simulink model "model"  (R2014a)
(part 2 of 3)

  _CN_244062688_500000_CN_163913701_500000 : powerlib/Elements/Distributed Parameters Line  Phases=3  Frequency=60  Resistance=[0.01273 0.3864]  Inductance="[0.9337e-3  4.1264e-3]"  Capacitance=[12.74e-9 7.751e-9]  Length=114.838  x1=[0 0 0 0; 0.0001244 0 0 0; 0.0002488 0 0 0; 0.0003733 0 0 0; 0.0004977 0 0 0; 0.0006221 0 0 0]  x2=[0 0 0 0; 0.0001244 0 0 0; 0.0002488 0 0 0; 0.0003733 0 0 0; 0.0004977 0 0 0; 0.0006221 0 0 0]  x3=[0 0 0 0; 0.0001244 0 0 0; 0.0002488 0 0 0; 0.0003733 0 0 0; 0.0004977 0 0 0; 0.0006221 0 0 0]  x4=[0 0 0 0; 0.0001244 0 0 0; 0.0002488 0 0 0; 0.0003733 0 0 0; 0.0004977 0 0 0; 0.0006221 0 0 0]  x5=0  V1=ones(3,3)  V2=ones(3,3)  I1=ones(3,3)  I2=ones(3,3)  nHarmo=1  Measurements=None
  _CN_255032299_110000_CN_255032301_110000 : powerlib/Elements/Distributed Parameters Line  Phases=3  Frequency=60  Resistance=[0.01273 0.3864]  Inductance="[0.9337e-3  4.1264e-3]"  Capacitance=[12.74e-9 7.751e-9]  Length=20.7716  x1=[0 0 0 0; 0.0001244 0 0 0; 0.0002488 0 0 0; 0.0003733 0 0 0; 0.0004977 0 0 0; 0.0006221 0 0 0]  x2=[0 0 0 0; 0.0001244 0 0 0; 0.0002488 0 0 0; 0.0003733 0 0 0; 0.0004977 0 0 0; 0.0006221 0 0 0]  x3=[0 0 0 0; 0.0001244 0 0 0; 0.0002488 0 0 0; 0.0003733 0 0 0; 0.0004977 0 0 0; 0.0006221 0 0 0]  x4=[0 0 0 0; 0.0001244 0 0 0; 0.0002488 0 0 0; 0.0003733 0 0 0; 0.0004977 0 0 0; 0.0006221 0 0 0]  x5=0  V1=ones(3,3)  V2=ones(3,3)  I1=ones(3,3)  I2=ones(3,3)  nHarmo=1  Measurements=None
  _CN_255624915_110000_CN_106927870_110000 : powerlib/Elements/Distributed Parameters Line  Phases=3  Frequency=60  Resistance=[0.01273 0.3864]  Inductance="[0.9337e-3  4.1264e-3]"  Capacitance=[12.74e-9 7.751e-9]  Length=19.6692  x1=[0 0 0 0; 0.0001244 0 0 0; 0.0002488 0 0 0; 0.0003733 0 0 0; 0.0004977 0 0 0; 0.0006221 0 0 0]  x2=[0 0 0 0; 0.0001244 0 0 0; 0.0002488 0 0 0; 0.0003733 0 0 0; 0.0004977 0 0 0; 0.0006221 0 0 0]  x3=[0 0 0 0; 0.0001244 0 0 0; 0.0002488 0 0 0; 0.0003733 0 0 0; 0.0004977 0 0 0; 0.0006221 0 0 0]  x4=[0 0 0 0; 0.0001244 0 0 0; 0.0002488 0 0 0; 0.0003733 0 0 0; 0.0004977 0 0 0; 0.0006221 0 0 0]  x5=0  V1=ones(3,3)  V2=ones(3,3)  I1=ones(3,3)  I2=ones(3,3)  nHarmo=1  Measurements=None
  _CN_266070665_110000_CN_130127057_110000 : powerlib/Elements/Distributed Parameters Line  Phases=3  Frequency=60  Resistance=[0.01273 0.3864]  Inductance="[0.9337e-3  4.1264e-3]"  Capacitance=[12.74e-9 7.751e-9]  Length=28.2359  x1=[0 0 0 0; 0.0001244 0 0 0; 0.0002488 0 0 0; 0.0003733 0 0 0; 0.0004977 0 0 0; 0.0006221 0 0 0]  x2=[0 0 0 0; 0.0001244 0 0 0; 0.0002488 0 0 0; 0.0003733 0 0 0; 0.0004977 0 0 0; 0.0006221 0 0 0]  x3=[0 0 0 0; 0.0001244 0 0 0; 0.0002488 0 0 0; 0.0003733 0 0 0; 0.0004977 0 0 0; 0.0006221 0 0 0]  x4=[0 0 0 0; 0.0001244 0 0 0; 0.0002488 0 0 0; 0.0003733 0 0 0; 0.0004977 0 0 0; 0.0006221 0 0 0]  x5=0  V1=ones(3,3)  V2=ones(3,3)  I1=ones(3,3)  I2=ones(3,3)  nHarmo=1  Measurements=None
  _CN_27258925_500000_CN_100289117_500000 : powerlib/Elements/Distributed Parameters Line  Phases=3  Frequency=60  Resistance=[0.01273 0.3864]  Inductance="[0.9337e-3  4.1264e-3]"  Capacitance=[12.74e-9 7.751e-9]  Length=52.4528  x1=[0 0 0 0; 0.0001244 0 0 0; 0.0002488 0 0 0; 0.0003733 0 0 0; 0.0004977 0 0 0; 0.0006221 0 0 0]  x2=[0 0 0 0; 0.0001244 0 0 0; 0.0002488 0 0 0; 0.0003733 0 0 0; 0.0004977 0 0 0; 0.0006221 0 0 0]  x3=[0 0 0 0; 0.0001244 0 0 0; 0.0002488 0 0 0; 0.0003733 0 0 0; 0.0004977 0 0 0; 0.0006221 0 0 0]  x4=[0 0 0 0; 0.0001244 0 0 0; 0.0002488 0 0 0; 0.0003733 0 0 0; 0.0004977 0 0 0; 0.0006221 0 0 0]  x5=0  V1=ones(3,3)  V2=ones(3,3)  I1=ones(3,3)  I2=ones(3,3)  nHarmo=1  Measurements=None
  _CN_27258925_500000_CN_159955044_220000 : powerlib/Elements/Distributed Parameters Line  Phases=3  Frequency=60  Resistance=[0.01273 0.3864]  Inductance="[0.9337e-3  4.1264e-3]"  Capacitance=[12.74e-9 7.751e-9]  Length=54.2482  x1=[0 0 0 0; 0.0001244 0 0 0; 0.0002488 0 0 0; 0.0003733 0 0 0; 0.0004977 0 0 0; 0.0006221 0 0 0]  x2=[0 0 0 0; 0.0001244 0 0 0; 0.0002488 0 0 0; 0.0003733 0 0 0; 0.0004977 0 0 0; 0.0006221 0 0 0]  x3=[0 0 0 0; 0.0001244 0 0 0; 0.0002488 0 0 0; 0.0003733 0 0 0; 0.0004977 0 0 0; 0.0006221 0 0 0]  x4=[0 0 0 0; 0.0001244 0 0 0; 0.0002488 0 0 0; 0.0003733 0 0 0; 0.0004977 0 0 0; 0.0006221 0 0 0]  x5=0  V1=ones(3,3)  V2=ones(3,3)  I1=ones(3,3)  I2=ones(3,3)  nHarmo=1  Measurements=None
  _CN_274652249_110000_CN_106927870_110000 : powerlib/Elements/Distributed Parameters Line  Phases=3  Frequency=60  Resistance=[0.01273 0.3864]  Inductance="[0.9337e-3  4.1264e-3]"  Capacitance=[12.74e-9 7.751e-9]  Length=20.7852  x1=[0 0 0 0; 0.0001244 0 0 0; 0.0002488 0 0 0; 0.0003733 0 0 0; 0.0004977 0 0 0; 0.0006221 0 0 0]  x2=[0 0 0 0; 0.0001244 0 0 0; 0.0002488 0 0 0; 0.0003733 0 0 0; 0.0004977 0 0 0; 0.0006221 0 0 0]  x3=[0 0 0 0; 0.0001244 0 0 0; 0.0002488 0 0 0; 0.0003733 0 0 0; 0.0004977 0 0 0; 0.0006221 0 0 0]  x4=[0 0 0 0; 0.0001244 0 0 0; 0.0002488 0 0 0; 0.0003733 0 0 0; 0.0004977 0 0 0; 0.0006221 0 0 0]  x5=0  V1=ones(3,3)  V2=ones(3,3)  I1=ones(3,3)  I2=ones(3,3)  nHarmo=1  Measurements=None
  _CN_274652249_110000_CN_216208030_110000 : powerlib/Elements/Distributed Parameters Line  Phases=3  Frequency=60  Resistance=[0.01273 0.3864]  Inductance="[0.9337e-3  4.1264e-3]"  Capacitance=[12.74e-9 7.751e-9]  Length=37.3748  x1=[0 0 0 0; 0.0001244 0 0 0; 0.0002488 0 0 0; 0.0003733 0 0 0; 0.0004977 0 0 0; 0.0006221 0 0 0]  x2=[0 0 0 0; 0.0001244 0 0 0; 0.0002488 0 0 0; 0.0003733 0 0 0; 0.0004977 0 0 0; 0.0006221 0 0 0]  x3=[0 0 0 0; 0.0001244 0 0 0; 0.0002488 0 0 0; 0.0003733 0 0 0; 0.0004977 0 0 0; 0.0006221 0 0 0]  x4=[0 0 0 0; 0.0001244 0 0 0; 0.0002488 0 0 0; 0.0003733 0 0 0; 0.0004977 0 0 0; 0.0006221 0 0 0]  x5=0  V1=ones(3,3)  V2=ones(3,3)  I1=ones(3,3)  I2=ones(3,3)  nHarmo=1  Measurements=None
  _CN_274652249_110000_CN_255624915_110000 : powerlib/Elements/Distributed Parameters Line  Phases=3  Frequency=60  Resistance=[0.01273 0.3864]  Inductance="[0.9337e-3  4.1264e-3]"  Capacitance=[12.74e-9 7.751e-9]  Length=40.3852  x1=[0 0 0 0; 0.0001244 0 0 0; 0.0002488 0 0 0; 0.0003733 0 0 0; 0.0004977 0 0 0; 0.0006221 0 0 0]  x2=[0 0 0 0; 0.0001244 0 0 0; 0.0002488 0 0 0; 0.0003733 0 0 0; 0.0004977 0 0 0; 0.0006221 0 0 0]  x3=[0 0 0 0; 0.0001244 0 0 0; 0.0002488 0 0 0; 0.0003733 0 0 0; 0.0004977 0 0 0; 0.0006221 0 0 0]  x4=[0 0 0 0; 0.0001244 0 0 0; 0.0002488 0 0 0; 0.0003733 0 0 0; 0.0004977 0 0 0; 0.0006221 0 0 0]  x5=0  V1=ones(3,3)  V2=ones(3,3)  I1=ones(3,3)  I2=ones(3,3)  nHarmo=1  Measurements=None
  _CN_275095874_220000_CN_93314614_220000 : powerlib/Elements/Distributed Parameters Line  Phases=3  Frequency=60  Resistance=[0.01273 0.3864]  Inductance="[0.9337e-3  4.1264e-3]"  Capacitance=[12.74e-9 7.751e-9]  Length=94.3159  x1=[0 0 0 0; 0.0001244 0 0 0; 0.0002488 0 0 0; 0.0003733 0 0 0; 0.0004977 0 0 0; 0.0006221 0 0 0]  x2=[0 0 0 0; 0.0001244 0 0 0; 0.0002488 0 0 0; 0.0003733 0 0 0; 0.0004977 0 0 0; 0.0006221 0 0 0]  x3=[0 0 0 0; 0.0001244 0 0 0; 0.0002488 0 0 0; 0.0003733 0 0 0; 0.0004977 0 0 0; 0.0006221 0 0 0]  x4=[0 0 0 0; 0.0001244 0 0 0; 0.0002488 0 0 0; 0.0003733 0 0 0; 0.0004977 0 0 0; 0.0006221 0 0 0]  x5=0  V1=ones(3,3)  V2=ones(3,3)  I1=ones(3,3)  I2=ones(3,3)  nHarmo=1  Measurements=None
  _CN_279497233_110000_CN_126093674_110000 : powerlib/Elements/Distributed Parameters Line  Phases=3  Frequency=60  Resistance=[0.01273 0.3864]  Inductance="[0.9337e-3  4.1264e-3]"  Capacitance=[12.74e-9 7.751e-9]  Length=30.1874  x1=[0 0 0 0; 0.0001244 0 0 0; 0.0002488 0 0 0; 0.0003733 0 0 0; 0.0004977 0 0 0; 0.0006221 0 0 0]  x2=[0 0 0 0; 0.0001244 0 0 0; 0.0002488 0 0 0; 0.0003733 0 0 0; 0.0004977 0 0 0; 0.0006221 0 0 0]  x3=[0 0 0 0; 0.0001244 0 0 0; 0.0002488 0 0 0; 0.0003733 0 0 0; 0.0004977 0 0 0; 0.0006221 0 0 0]  x4=[0 0 0 0; 0.0001244 0 0 0; 0.0002488 0 0 0; 0.0003733 0 0 0; 0.0004977 0 0 0; 0.0006221 0 0 0]  x5=0  V1=ones(3,3)  V2=ones(3,3)  I1=ones(3,3)  I2=ones(3,3)  nHarmo=1  Measurements=None
  _CN_280421437_110000_CN_166188874_110000 : powerlib/Elements/Distributed Parameters Line  Phases=3  Frequency=60  Resistance=[0.01273 0.3864]  Inductance="[0.9337e-3  4.1264e-3]"  Capacitance=[12.74e-9 7.751e-9]  Length=1.4097  x1=[0 0 0 0; 0.0001244 0 0 0; 0.0002488 0 0 0; 0.0003733 0 0 0; 0.0004977 0 0 0; 0.0006221 0 0 0]  x2=[0 0 0 0; 0.0001244 0 0 0; 0.0002488 0 0 0; 0.0003733 0 0 0; 0.0004977 0 0 0; 0.0006221 0 0 0]  x3=[0 0 0 0; 0.0001244 0 0 0; 0.0002488 0 0 0; 0.0003733 0 0 0; 0.0004977 0 0 0; 0.0006221 0 0 0]  x4=[0 0 0 0; 0.0001244 0 0 0; 0.0002488 0 0 0; 0.0003733 0 0 0; 0.0004977 0 0 0; 0.0006221 0 0 0]  x5=0  V1=ones(3,3)  V2=ones(3,3)  I1=ones(3,3)  I2=ones(3,3)  nHarmo=1  Measurements=None
  _CN_282645278_110000_CN_166188874_110000 : powerlib/Elements/Distributed Parameters Line  Phases=3  Frequency=60  Resistance=[0.01273 0.3864]  Inductance="[0.9337e-3  4.1264e-3]"  Capacitance=[12.74e-9 7.751e-9]  Length=5.961  x1=[0 0 0 0; 0.0001244 0 0 0; 0.0002488 0 0 0; 0.0003733 0 0 0; 0.0004977 0 0 0; 0.0006221 0 0 0]  x2=[0 0 0 0; 0.0001244 0 0 0; 0.0002488 0 0 0; 0.0003733 0 0 0; 0.0004977 0 0 0; 0.0006221 0 0 0]  x3=[0 0 0 0; 0.0001244 0 0 0; 0.0002488 0 0 0; 0.0003733 0 0 0; 0.0004977 0 0 0; 0.0006221 0 0 0]  x4=[0 0 0 0; 0.0001244 0 0 0; 0.0002488 0 0 0; 0.0003733 0 0 0; 0.0004977 0 0 0; 0.0006221 0 0 0]  x5=0  V1=ones(3,3)  V2=ones(3,3)  I1=ones(3,3)  I2=ones(3,3)  nHarmo=1  Measurements=None
  _CN_282779585_110000_CN_282779587_110000 : powerlib/Elements/Distributed Parameters Line  Phases=3  Frequency=60  Resistance=[0.01273 0.3864]  Inductance="[0.9337e-3  4.1264e-3]"  Capacitance=[12.74e-9 7.751e-9]  Length=0.85619  x1=[0 0 0 0; 0.0001244 0 0 0; 0.0002488 0 0 0; 0.0003733 0 0 0; 0.0004977 0 0 0; 0.0006221 0 0 0]  x2=[0 0 0 0; 0.0001244 0 0 0; 0.0002488 0 0 0; 0.0003733 0 0 0; 0.0004977 0 0 0; 0.0006221 0 0 0]  x3=[0 0 0 0; 0.0001244 0 0 0; 0.0002488 0 0 0; 0.0003733 0 0 0; 0.0004977 0 0 0; 0.0006221 0 0 0]  x4=[0 0 0 0; 0.0001244 0 0 0; 0.0002488 0 0 0; 0.0003733 0 0 0; 0.0004977 0 0 0; 0.0006221 0 0 0]  x5=0  V1=ones(3,3)  V2=ones(3,3)  I1=ones(3,3)  I2=ones(3,3)  nHarmo=1  Measurements=None
  _CN_282779585_110000_CN_93418566_110000 : powerlib/Elements/Distributed Parameters Line  Phases=3  Frequency=60  Resistance=[0.01273 0.3864]  Inductance="[0.9337e-3  4.1264e-3]"  Capacitance=[12.74e-9 7.751e-9]  Length=7.1591  x1=[0 0 0 0; 0.0001244 0 0 0; 0.0002488 0 0 0; 0.0003733 0 0 0; 0.0004977 0 0 0; 0.0006221 0 0 0]  x2=[0 0 0 0; 0.0001244 0 0 0; 0.0002488 0 0 0; 0.0003733 0 0 0; 0.0004977 0 0 0; 0.0006221 0 0 0]  x3=[0 0 0 0; 0.0001244 0 0 0; 0.0002488 0 0 0; 0.0003733 0 0 0; 0.0004977 0 0 0; 0.0006221 0 0 0]  x4=[0 0 0 0; 0.0001244 0 0 0; 0.0002488 0 0 0; 0.0003733 0 0 0; 0.0004977 0 0 0; 0.0006221 0 0 0]  x5=0  V1=ones(3,3)  V2=ones(3,3)  I1=ones(3,3)  I2=ones(3,3)  nHarmo=1  Measurements=None
  _CN_282779592_110000_CN_92045303_110000 : powerlib/Elements/Distributed Parameters Line  Phases=3  Frequency=60  Resistance=[0.01273 0.3864]  Inductance="[0.9337e-3  4.1264e-3]"  Capacitance=[12.74e-9 7.751e-9]  Length=6.7197  x1=[0 0 0 0; 0.0001244 0 0 0; 0.0002488 0 0 0; 0.0003733 0 0 0; 0.0004977 0 0 0; 0.0006221 0 0 0]  x2=[0 0 0 0; 0.0001244 0 0 0; 0.0002488 0 0 0; 0.0003733 0 0 0; 0.0004977 0 0 0; 0.0006221 0 0 0]  x3=[0 0 0 0; 0.0001244 0 0 0; 0.0002488 0 0 0; 0.0003733 0 0 0; 0.0004977 0 0 0; 0.0006221 0 0 0]  x4=[0 0 0 0; 0.0001244 0 0 0; 0.0002488 0 0 0; 0.0003733 0 0 0; 0.0004977 0 0 0; 0.0006221 0 0 0]  x5=0  V1=ones(3,3)  V2=ones(3,3)  I1=ones(3,3)  I2=ones(3,3)  nHarmo=1  Measurements=None
  _CN_286951577_110000_CN_116299140_110000 : powerlib/Elements/Distributed Parameters Line  Phases=3  Frequency=60  Resistance=[0.01273 0.3864]  Inductance="[0.9337e-3  4.1264e-3]"  Capacitance=[12.74e-9 7.751e-9]  Length=25.7872  x1=[0 0 0 0; 0.0001244 0 0 0; 0.0002488 0 0 0; 0.0003733 0 0 0; 0.0004977 0 0 0; 0.0006221 0 0 0]  x2=[0 0 0 0; 0.0001244 0 0 0; 0.0002488 0 0 0; 0.0003733 0 0 0; 0.0004977 0 0 0; 0.0006221 0 0 0]  x3=[0 0 0 0; 0.0001244 0 0 0; 0.0002488 0 0 0; 0.0003733 0 0 0; 0.0004977 0 0 0; 0.0006221 0 0 0]  x4=[0 0 0 0; 0.0001244 0 0 0; 0.0002488 0 0 0; 0.0003733 0 0 0; 0.0004977 0 0 0; 0.0006221 0 0 0]  x5=0  V1=ones(3,3)  V2=ones(3,3)  I1=ones(3,3)  I2=ones(3,3)  nHarmo=1  Measurements=None
  _CN_305096727_110000_CN_354777580_110000 : powerlib/Elements/Distributed Parameters Line  Phases=3  Frequency=60  Resistance=[0.01273 0.3864]  Inductance="[0.9337e-3  4.1264e-3]"  Capacitance=[12.74e-9 7.751e-9]  Length=16.9581  x1=[0 0 0 0; 0.0001244 0 0 0; 0.0002488 0 0 0; 0.0003733 0 0 0; 0.0004977 0 0 0; 0.0006221 0 0 0]  x2=[0 0 0 0; 0.0001244 0 0 0; 0.0002488 0 0 0; 0.0003733 0 0 0; 0.0004977 0 0 0; 0.0006221 0 0 0]  x3=[0 0 0 0; 0.0001244 0 0 0; 0.0002488 0 0 0; 0.0003733 0 0 0; 0.0004977 0 0 0; 0.0006221 0 0 0]  x4=[0 0 0 0; 0.0001244 0 0 0; 0.0002488 0 0 0; 0.0003733 0 0 0; 0.0004977 0 0 0; 0.0006221 0 0 0]  x5=0  V1=ones(3,3)  V2=ones(3,3)  I1=ones(3,3)  I2=ones(3,3)  nHarmo=1  Measurements=None
  _CN_306102396_110000_CN_305096727_110000 : powerlib/Elements/Distributed Parameters Line  Phases=3  Frequency=60  Resistance=[0.01273 0.3864]  Inductance="[0.9337e-3  4.1264e-3]"  Capacitance=[12.74e-9 7.751e-9]  Length=15.5705  x1=[0 0 0 0; 0.0001244 0 0 0; 0.0002488 0 0 0; 0.0003733 0 0 0; 0.0004977 0 0 0; 0.0006221 0 0 0]  x2=[0 0 0 0; 0.0001244 0 0 0; 0.0002488 0 0 0; 0.0003733 0 0 0; 0.0004977 0 0 0; 0.0006221 0 0 0]  x3=[0 0 0 0; 0.0001244 0 0 0; 0.0002488 0 0 0; 0.0003733 0 0 0; 0.0004977 0 0 0; 0.0006221 0 0 0]  x4=[0 0 0 0; 0.0001244 0 0 0; 0.0002488 0 0 0; 0.0003733 0 0 0; 0.0004977 0 0 0; 0.0006221 0 0 0]  x5=0  V1=ones(3,3)  V2=ones(3,3)  I1=ones(3,3)  I2=ones(3,3)  nHarmo=1  Measurements=None
  _CN_320347053_110000_CN_93050981_110000 : powerlib/Elements/Distributed Parameters Line  Phases=3  Frequency=60  Resistance=[0.01273 0.3864]  Inductance="[0.9337e-3  4.1264e-3]"  Capacitance=[12.74e-9 7.751e-9]  Length=30.0393  x1=[0 0 0 0; 0.0001244 0 0 0; 0.0002488 0 0 0; 0.0003733 0 0 0; 0.0004977 0 0 0; 0.0006221 0 0 0]  x2=[0 0 0 0; 0.0001244 0 0 0; 0.0002488 0 0 0; 0.0003733 0 0 0; 0.0004977 0 0 0; 0.0006221 0 0 0]  x3=[0 0 0 0; 0.0001244 0 0 0; 0.0002488 0 0 0; 0.0003733 0 0 0; 0.0004977 0 0 0; 0.0006221 0 0 0]  x4=[0 0 0 0; 0.0001244 0 0 0; 0.0002488 0 0 0; 0.0003733 0 0 0; 0.0004977 0 0 0; 0.0006221 0 0 0]  x5=0  V1=ones(3,3)  V2=ones(3,3)  I1=ones(3,3)  I2=ones(3,3)  nHarmo=1  Measurements=None
  _CN_325873379_110000_CN_90797306_110000 : powerlib/Elements/Distributed Parameters Line  Phases=3  Frequency=60  Resistance=[0.01273 0.3864]  Inductance="[0.9337e-3  4.1264e-3]"  Capacitance=[12.74e-9 7.751e-9]  Length=7.1372  x1=[0 0 0 0; 0.0001244 0 0 0; 0.0002488 0 0 0; 0.0003733 0 0 0; 0.0004977 0 0 0; 0.0006221 0 0 0]  x2=[0 0 0 0; 0.0001244 0 0 0; 0.0002488 0 0 0; 0.0003733 0 0 0; 0.0004977 0 0 0; 0.0006221 0 0 0]  x3=[0 0 0 0; 0.0001244 0 0 0; 0.0002488 0 0 0; 0.0003733 0 0 0; 0.0004977 0 0 0; 0.0006221 0 0 0]  x4=[0 0 0 0; 0.0001244 0 0 0; 0.0002488 0 0 0; 0.0003733 0 0 0; 0.0004977 0 0 0; 0.0006221 0 0 0]  x5=0  V1=ones(3,3)  V2=ones(3,3)  I1=ones(3,3)  I2=ones(3,3)  nHarmo=1  Measurements=None
  _CN_331102892_110000_CN_128346488_110000 : powerlib/Elements/Distributed Parameters Line  Phases=3  Frequency=60  Resistance=[0.01273 0.3864]  Inductance="[0.9337e-3  4.1264e-3]"  Capacitance=[12.74e-9 7.751e-9]  Length=7.8937  x1=[0 0 0 0; 0.0001244 0 0 0; 0.0002488 0 0 0; 0.0003733 0 0 0; 0.0004977 0 0 0; 0.0006221 0 0 0]  x2=[0 0 0 0; 0.0001244 0 0 0; 0.0002488 0 0 0; 0.0003733 0 0 0; 0.0004977 0 0 0; 0.0006221 0 0 0]  x3=[0 0 0 0; 0.0001244 0 0 0; 0.0002488 0 0 0; 0.0003733 0 0 0; 0.0004977 0 0 0; 0.0006221 0 0 0]  x4=[0 0 0 0; 0.0001244 0 0 0; 0.0002488 0 0 0; 0.0003733 0 0 0; 0.0004977 0 0 0; 0.0006221 0 0 0]  x5=0  V1=ones(3,3)  V2=ones(3,3)  I1=ones(3,3)  I2=ones(3,3)  nHarmo=1  Measurements=None
  _CN_331102892_110000_CN_164371995_110000 : powerlib/Elements/Distributed Parameters Line  Phases=3  Frequency=60  Resistance=[0.01273 0.3864]  Inductance="[0.9337e-3  4.1264e-3]"  Capacitance=[12.74e-9 7.751e-9]  Length=27.0823  x1=[0 0 0 0; 0.0001244 0 0 0; 0.0002488 0 0 0; 0.0003733 0 0 0; 0.0004977 0 0 0; 0.0006221 0 0 0]  x2=[0 0 0 0; 0.0001244 0 0 0; 0.0002488 0 0 0; 0.0003733 0 0 0; 0.0004977 0 0 0; 0.0006221 0 0 0]  x3=[0 0 0 0; 0.0001244 0 0 0; 0.0002488 0 0 0; 0.0003733 0 0 0; 0.0004977 0 0 0; 0.0006221 0 0 0]  x4=[0 0 0 0; 0.0001244 0 0 0; 0.0002488 0 0 0; 0.0003733 0 0 0; 0.0004977 0 0 0; 0.0006221 0 0 0]  x5=0  V1=ones(3,3)  V2=ones(3,3)  I1=ones(3,3)  I2=ones(3,3)  nHarmo=1  Measurements=None
  _CN_331102892_110000_CN_187971431_110000 : powerlib/Elements/Distributed Parameters Line  Phases=3  Frequency=60  Resistance=[0.01273 0.3864]  Inductance="[0.9337e-3  4.1264e-3]"  Capacitance=[12.74e-9 7.751e-9]  Length=34.1401  x1=[0 0 0 0; 0.0001244 0 0 0; 0.0002488 0 0 0; 0.0003733 0 0 0; 0.0004977 0 0 0; 0.0006221 0 0 0]  x2=[0 0 0 0; 0.0001244 0 0 0; 0.0002488 0 0 0; 0.0003733 0 0 0; 0.0004977 0 0 0; 0.0006221 0 0 0]  x3=[0 0 0 0; 0.0001244 0 0 0; 0.0002488 0 0 0; 0.0003733 0 0 0; 0.0004977 0 0 0; 0.0006221 0 0 0]  x4=[0 0 0 0; 0.0001244 0 0 0; 0.0002488 0 0 0; 0.0003733 0 0 0; 0.0004977 0 0 0; 0.0006221 0 0 0]  x5=0  V1=ones(3,3)  V2=ones(3,3)  I1=ones(3,3)  I2=ones(3,3)  nHarmo=1  Measurements=None
  _CN_331102892_110000_CN_93050981_110000 : powerlib/Elements/Distributed Parameters Line  Phases=3  Frequency=60  Resistance=[0.01273 0.3864]  Inductance="[0.9337e-3  4.1264e-3]"  Capacitance=[12.74e-9 7.751e-9]  Length=34.1134  x1=[0 0 0 0; 0.0001244 0 0 0; 0.0002488 0 0 0; 0.0003733 0 0 0; 0.0004977 0 0 0; 0.0006221 0 0 0]  x2=[0 0 0 0; 0.0001244 0 0 0; 0.0002488 0 0 0; 0.0003733 0 0 0; 0.0004977 0 0 0; 0.0006221 0 0 0]  x3=[0 0 0 0; 0.0001244 0 0 0; 0.0002488 0 0 0; 0.0003733 0 0 0; 0.0004977 0 0 0; 0.0006221 0 0 0]  x4=[0 0 0 0; 0.0001244 0 0 0; 0.0002488 0 0 0; 0.0003733 0 0 0; 0.0004977 0 0 0; 0.0006221 0 0 0]  x5=0  V1=ones(3,3)  V2=ones(3,3)  I1=ones(3,3)  I2=ones(3,3)  nHarmo=1  Measurements=None
  _CN_332377360_110000_CN_354777580_110000 : powerlib/Elements/Distributed Parameters Line  Phases=3  Frequency=60  Resistance=[0.01273 0.3864]  Inductance="[0.9337e-3  4.1264e-3]"  Capacitance=[12.74e-9 7.751e-9]  Length=17.4914  x1=[0 0 0 0; 0.0001244 0 0 0; 0.0002488 0 0 0; 0.0003733 0 0 0; 0.0004977 0 0 0; 0.0006221 0 0 0]  x2=[0 0 0 0; 0.0001244 0 0 0; 0.0002488 0 0 0; 0.0003733 0 0 0; 0.0004977 0 0 0; 0.0006221 0 0 0]  x3=[0 0 0 0; 0.0001244 0 0 0; 0.0002488 0 0 0; 0.0003733 0 0 0; 0.0004977 0 0 0; 0.0006221 0 0 0]  x4=[0 0 0 0; 0.0001244 0 0 0; 0.0002488 0 0 0; 0.0003733 0 0 0; 0.0004977 0 0 0; 0.0006221 0 0 0]  x5=0  V1=ones(3,3)  V2=ones(3,3)  I1=ones(3,3)  I2=ones(3,3)  nHarmo=1  Measurements=None
  _CN_337947383_110000_CN_220103258_110000 : powerlib/Elements/Distributed Parameters Line  Phases=3  Frequency=60  Resistance=[0.01273 0.3864]  Inductance="[0.9337e-3  4.1264e-3]"  Capacitance=[12.74e-9 7.751e-9]  Length=1.5396  x1=[0 0 0 0; 0.0001244 0 0 0; 0.0002488 0 0 0; 0.0003733 0 0 0; 0.0004977 0 0 0; 0.0006221 0 0 0]  x2=[0 0 0 0; 0.0001244 0 0 0; 0.0002488 0 0 0; 0.0003733 0 0 0; 0.0004977 0 0 0; 0.0006221 0 0 0]  x3=[0 0 0 0; 0.0001244 0 0 0; 0.0002488 0 0 0; 0.0003733 0 0 0; 0.0004977 0 0 0; 0.0006221 0 0 0]  x4=[0 0 0 0; 0.0001244 0 0 0; 0.0002488 0 0 0; 0.0003733 0 0 0; 0.0004977 0 0 0; 0.0006221 0 0 0]  x5=0  V1=ones(3,3)  V2=ones(3,3)  I1=ones(3,3)  I2=ones(3,3)  nHarmo=1  Measurements=None
  _CN_349543035_220000_CN_68522408_220000 : powerlib/Elements/Distributed Parameters Line  Phases=3  Frequency=60  Resistance=[0.01273 0.3864]  Inductance="[0.9337e-3  4.1264e-3]"  Capacitance=[12.74e-9 7.751e-9]  Length=24.4426  x1=[0 0 0 0; 0.0001244 0 0 0; 0.0002488 0 0 0; 0.0003733 0 0 0; 0.0004977 0 0 0; 0.0006221 0 0 0]  x2=[0 0 0 0; 0.0001244 0 0 0; 0.0002488 0 0 0; 0.0003733 0 0 0; 0.0004977 0 0 0; 0.0006221 0 0 0]  x3=[0 0 0 0; 0.0001244 0 0 0; 0.0002488 0 0 0; 0.0003733 0 0 0; 0.0004977 0 0 0; 0.0006221 0 0 0]  x4=[0 0 0 0; 0.0001244 0 0 0; 0.0002488 0 0 0; 0.0003733 0 0 0; 0.0004977 0 0 0; 0.0006221 0 0 0]  x5=0  V1=ones(3,3)  V2=ones(3,3)  I1=ones(3,3)  I2=ones(3,3)  nHarmo=1  Measurements=None
  _CN_352282301_110000_CN_138410290_110000 : powerlib/Elements/Distributed Parameters Line  Phases=3  Frequency=60  Resistance=[0.01273 0.3864]  Inductance="[0.9337e-3  4.1264e-3]"  Capacitance=[12.74e-9 7.751e-9]  Length=27.3015  x1=[0 0 0 0; 0.0001244 0 0 0; 0.0002488 0 0 0; 0.0003733 0 0 0; 0.0004977 0 0 0; 0.0006221 0 0 0]  x2=[0 0 0 0; 0.0001244 0 0 0; 0.0002488 0 0 0; 0.0003733 0 0 0; 0.0004977 0 0 0; 0.0006221 0 0 0]  x3=[0 0 0 0; 0.0001244 0 0 0; 0.0002488 0 0 0; 0.0003733 0 0 0; 0.0004977 0 0 0; 0.0006221 0 0 0]  x4=[0 0 0 0; 0.0001244 0 0 0; 0.0002488 0 0 0; 0.0003733 0 0 0; 0.0004977 0 0 0; 0.0006221 0 0 0]  x5=0  V1=ones(3,3)  V2=ones(3,3)  I1=ones(3,3)  I2=ones(3,3)  nHarmo=1  Measurements=None
  _CN_361264295_110000_CN_116299140_110000 : powerlib/Elements/Distributed Parameters Line  Phases=3  Frequency=60  Resistance=[0.01273 0.3864]  Inductance="[0.9337e-3  4.1264e-3]"  Capacitance=[12.74e-9 7.751e-9]  Length=14.4602  x1=[0 0 0 0; 0.0001244 0 0 0; 0.0002488 0 0 0; 0.0003733 0 0 0; 0.0004977 0 0 0; 0.0006221 0 0 0]  x2=[0 0 0 0; 0.0001244 0 0 0; 0.0002488 0 0 0; 0.0003733 0 0 0; 0.0004977 0 0 0; 0.0006221 0 0 0]  x3=[0 0 0 0; 0.0001244 0 0 0; 0.0002488 0 0 0; 0.0003733 0 0 0; 0.0004977 0 0 0; 0.0006221 0 0 0]  x4=[0 0 0 0; 0.0001244 0 0 0; 0.0002488 0 0 0; 0.0003733 0 0 0; 0.0004977 0 0 0; 0.0006221 0 0 0]  x5=0  V1=ones(3,3)  V2=ones(3,3)  I1=ones(3,3)  I2=ones(3,3)  nHarmo=1  Measurements=None
  _CN_361264295_110000_CN_372580522_110000 : powerlib/Elements/Distributed Parameters Line  Phases=3  Frequency=60  Resistance=[0.01273 0.3864]  Inductance="[0.9337e-3  4.1264e-3]"  Capacitance=[12.74e-9 7.751e-9]  Length=30.4838  x1=[0 0 0 0; 0.0001244 0 0 0; 0.0002488 0 0 0; 0.0003733 0 0 0; 0.0004977 0 0 0; 0.0006221 0 0 0]  x2=[0 0 0 0; 0.0001244 0 0 0; 0.0002488 0 0 0; 0.0003733 0 0 0; 0.0004977 0 0 0; 0.0006221 0 0 0]  x3=[0 0 0 0; 0.0001244 0 0 0; 0.0002488 0 0 0; 0.0003733 0 0 0; 0.0004977 0 0 0; 0.0006221 0 0 0]  x4=[0 0 0 0; 0.0001244 0 0 0; 0.0002488 0 0 0; 0.0003733 0 0 0; 0.0004977 0 0 0; 0.0006221 0 0 0]  x5=0  V1=ones(3,3)  V2=ones(3,3)  I1=ones(3,3)  I2=ones(3,3)  nHarmo=1  Measurements=None
  _CN_361265069_110000_CN_116299140_110000 : powerlib/Elements/Distributed Parameters Line  Phases=3  Frequency=60  Resistance=[0.01273 0.3864]  Inductance="[0.9337e-3  4.1264e-3]"  Capacitance=[12.74e-9 7.751e-9]  Length=1.5824  x1=[0 0 0 0; 0.0001244 0 0 0; 0.0002488 0 0 0; 0.0003733 0 0 0; 0.0004977 0 0 0; 0.0006221 0 0 0]  x2=[0 0 0 0; 0.0001244 0 0 0; 0.0002488 0 0 0; 0.0003733 0 0 0; 0.0004977 0 0 0; 0.0006221 0 0 0]  x3=[0 0 0 0; 0.0001244 0 0 0; 0.0002488 0 0 0; 0.0003733 0 0 0; 0.0004977 0 0 0; 0.0006221 0 0 0]  x4=[0 0 0 0; 0.0001244 0 0 0; 0.0002488 0 0 0; 0.0003733 0 0 0; 0.0004977 0 0 0; 0.0006221 0 0 0]  x5=0  V1=ones(3,3)  V2=ones(3,3)  I1=ones(3,3)  I2=ones(3,3)  nHarmo=1  Measurements=None
  _CN_361266572_110000_CN_116299140_110000 : powerlib/Elements/Distributed Parameters Line  Phases=3  Frequency=60  Resistance=[0.01273 0.3864]  Inductance="[0.9337e-3  4.1264e-3]"  Capacitance=[12.74e-9 7.751e-9]  Length=3.3962  x1=[0 0 0 0; 0.0001244 0 0 0; 0.0002488 0 0 0; 0.0003733 0 0 0; 0.0004977 0 0 0; 0.0006221 0 0 0]  x2=[0 0 0 0; 0.0001244 0 0 0; 0.0002488 0 0 0; 0.0003733 0 0 0; 0.0004977 0 0 0; 0.0006221 0 0 0]  x3=[0 0 0 0; 0.0001244 0 0 0; 0.0002488 0 0 0; 0.0003733 0 0 0; 0.0004977 0 0 0; 0.0006221 0 0 0]  x4=[0 0 0 0; 0.0001244 0 0 0; 0.0002488 0 0 0; 0.0003733 0 0 0; 0.0004977 0 0 0; 0.0006221 0 0 0]  x5=0  V1=ones(3,3)  V2=ones(3,3)  I1=ones(3,3)  I2=ones(3,3)  nHarmo=1  Measurements=None
  _CN_372580506_110000_CN_98423617_110000 : powerlib/Elements/Distributed Parameters Line  Phases=3  Frequency=60  Resistance=[0.01273 0.3864]  Inductance="[0.9337e-3  4.1264e-3]"  Capacitance=[12.74e-9 7.751e-9]  Length=43.9758  x1=[0 0 0 0; 0.0001244 0 0 0; 0.0002488 0 0 0; 0.0003733 0 0 0; 0.0004977 0 0 0; 0.0006221 0 0 0]  x2=[0 0 0 0; 0.0001244 0 0 0; 0.0002488 0 0 0; 0.0003733 0 0 0; 0.0004977 0 0 0; 0.0006221 0 0 0]  x3=[0 0 0 0; 0.0001244 0 0 0; 0.0002488 0 0 0; 0.0003733 0 0 0; 0.0004977 0 0 0; 0.0006221 0 0 0]  x4=[0 0 0 0; 0.0001244 0 0 0; 0.0002488 0 0 0; 0.0003733 0 0 0; 0.0004977 0 0 0; 0.0006221 0 0 0]  x5=0  V1=ones(3,3)  V2=ones(3,3)  I1=ones(3,3)  I2=ones(3,3)  nHarmo=1  Measurements=None
  _CN_386978254_110000_CN_163401683_110000 : powerlib/Elements/Distributed Parameters Line  Phases=3  Frequency=60  Resistance=[0.01273 0.3864]  Inductance="[0.9337e-3  4.1264e-3]"  Capacitance=[12.74e-9 7.751e-9]  Length=62.4742  x1=[0 0 0 0; 0.0001244 0 0 0; 0.0002488 0 0 0; 0.0003733 0 0 0; 0.0004977 0 0 0; 0.0006221 0 0 0]  x2=[0 0 0 0; 0.0001244 0 0 0; 0.0002488 0 0 0; 0.0003733 0 0 0; 0.0004977 0 0 0; 0.0006221 0 0 0]  x3=[0 0 0 0; 0.0001244 0 0 0; 0.0002488 0 0 0; 0.0003733 0 0 0; 0.0004977 0 0 0; 0.0006221 0 0 0]  x4=[0 0 0 0; 0.0001244 0 0 0; 0.0002488 0 0 0; 0.0003733 0 0 0; 0.0004977 0 0 0; 0.0006221 0 0 0]  x5=0  V1=ones(3,3)  V2=ones(3,3)  I1=ones(3,3)  I2=ones(3,3)  nHarmo=1  Measurements=None
  _CN_41528780_500000_CN_169556579_500000 : powerlib/Elements/Distributed Parameters Line  Phases=3  Frequency=60  Resistance=[0.01273 0.3864]  Inductance="[0.9337e-3  4.1264e-3]"  Capacitance=[12.74e-9 7.751e-9]  Length=44.3156  x1=[0 0 0 0; 0.0001244 0 0 0; 0.0002488 0 0 0; 0.0003733 0 0 0; 0.0004977 0 0 0; 0.0006221 0 0 0]  x2=[0 0 0 0; 0.0001244 0 0 0; 0.0002488 0 0 0; 0.0003733 0 0 0; 0.0004977 0 0 0; 0.0006221 0 0 0]  x3=[0 0 0 0; 0.0001244 0 0 0; 0.0002488 0 0 0; 0.0003733 0 0 0; 0.0004977 0 0 0; 0.0006221 0 0 0]  x4=[0 0 0 0; 0.0001244 0 0 0; 0.0002488 0 0 0; 0.0003733 0 0 0; 0.0004977 0 0 0; 0.0006221 0 0 0]  x5=0  V1=ones(3,3)  V2=ones(3,3)  I1=ones(3,3)  I2=ones(3,3)  nHarmo=1  Measurements=None
  _CN_81131204_220000_CN_150165502_220000 : powerlib/Elements/Distributed Parameters Line  Phases=3  Frequency=60  Resistance=[0.01273 0.3864]  Inductance="[0.9337e-3  4.1264e-3]"  Capacitance=[12.74e-9 7.751e-9]  Length=9.1709  x1=[0 0 0 0; 0.0001244 0 0 0; 0.0002488 0 0 0; 0.0003733 0 0 0; 0.0004977 0 0 0; 0.0006221 0 0 0]  x2=[0 0 0 0; 0.0001244 0 0 0; 0.0002488 0 0 0; 0.0003733 0 0 0; 0.0004977 0 0 0; 0.0006221 0 0 0]  x3=[0 0 0 0; 0.0001244 0 0 0; 0.0002488 0 0 0; 0.0003733 0 0 0; 0.0004977 0 0 0; 0.0006221 0 0 0]  x4=[0 0 0 0; 0.0001244 0 0 0; 0.0002488 0 0 0; 0.0003733 0 0 0; 0.0004977 0 0 0; 0.0006221 0 0 0]  x5=0  V1=ones(3,3)  V2=ones(3,3)  I1=ones(3,3)  I2=ones(3,3)  nHarmo=1  Measurements=None
  _CN_85603217_220000_CN_159955044_220000 : powerlib/Elements/Distributed Parameters Line  Phases=3  Frequency=60  Resistance=[0.01273 0.3864]  Inductance="[0.9337e-3  4.1264e-3]"  Capacitance=[12.74e-9 7.751e-9]  Length=34.2821  x1=[0 0 0 0; 0.0001244 0 0 0; 0.0002488 0 0 0; 0.0003733 0 0 0; 0.0004977 0 0 0; 0.0006221 0 0 0]  x2=[0 0 0 0; 0.0001244 0 0 0; 0.0002488 0 0 0; 0.0003733 0 0 0; 0.0004977 0 0 0; 0.0006221 0 0 0]  x3=[0 0 0 0; 0.0001244 0 0 0; 0.0002488 0 0 0; 0.0003733 0 0 0; 0.0004977 0 0 0; 0.0006221 0 0 0]  x4=[0 0 0 0; 0.0001244 0 0 0; 0.0002488 0 0 0; 0.0003733 0 0 0; 0.0004977 0 0 0; 0.0006221 0 0 0]  x5=0  V1=ones(3,3)  V2=ones(3,3)  I1=ones(3,3)  I2=ones(3,3)  nHarmo=1  Measurements=None
  _CN_93314614_220000_CN_96040535_220000 : powerlib/Elements/Distributed Parameters Line  Phases=3  Frequency=60  Resistance=[0.01273 0.3864]  Inductance="[0.9337e-3  4.1264e-3]"  Capacitance=[12.74e-9 7.751e-9]  Length=17.2248  x1=[0 0 0 0; 0.0001244 0 0 0; 0.0002488 0 0 0; 0.0003733 0 0 0; 0.0004977 0 0 0; 0.0006221 0 0 0]  x2=[0 0 0 0; 0.0001244 0 0 0; 0.0002488 0 0 0; 0.0003733 0 0 0; 0.0004977 0 0 0; 0.0006221 0 0 0]  x3=[0 0 0 0; 0.0001244 0 0 0; 0.0002488 0 0 0; 0.0003733 0 0 0; 0.0004977 0 0 0; 0.0006221 0 0 0]  x4=[0 0 0 0; 0.0001244 0 0 0; 0.0002488 0 0 0; 0.0003733 0 0 0; 0.0004977 0 0 0; 0.0006221 0 0 0]  x5=0  V1=ones(3,3)  V2=ones(3,3)  I1=ones(3,3)  I2=ones(3,3)  nHarmo=1  Measurements=None
  _CN_93314614_500000_CN_159955044_220000 : powerlib/Elements/Distributed Parameters Line  Phases=3  Frequency=60  Resistance=[0.01273 0.3864]  Inductance="[0.9337e-3  4.1264e-3]"  Capacitance=[12.74e-9 7.751e-9]  Length=135.2697  x1=[0 0 0 0; 0.0001244 0 0 0; 0.0002488 0 0 0; 0.0003733 0 0 0; 0.0004977 0 0 0; 0.0006221 0 0 0]  x2=[0 0 0 0; 0.0001244 0 0 0; 0.0002488 0 0 0; 0.0003733 0 0 0; 0.0004977 0 0 0; 0.0006221 0 0 0]  x3=[0 0 0 0; 0.0001244 0 0 0; 0.0002488 0 0 0; 0.0003733 0 0 0; 0.0004977 0 0 0; 0.0006221 0 0 0]  x4=[0 0 0 0; 0.0001244 0 0 0; 0.0002488 0 0 0; 0.0003733 0 0 0; 0.0004977 0 0 0; 0.0006221 0 0 0]  x5=0  V1=ones(3,3)  V2=ones(3,3)  I1=ones(3,3)  I2=ones(3,3)  nHarmo=1  Measurements=None
  _CN_93418566_110000_CN_166188874_110000 : powerlib/Elements/Distributed Parameters Line  Phases=3  Frequency=60  Resistance=[0.01273 0.3864]  Inductance="[0.9337e-3  4.1264e-3]"  Capacitance=[12.74e-9 7.751e-9]  Length=6.4317  x1=[0 0 0 0; 0.0001244 0 0 0; 0.0002488 0 0 0; 0.0003733 0 0 0; 0.0004977 0 0 0; 0.0006221 0 0 0]  x2=[0 0 0 0; 0.0001244 0 0 0; 0.0002488 0 0 0; 0.0003733 0 0 0; 0.0004977 0 0 0; 0.0006221 0 0 0]  x3=[0 0 0 0; 0.0001244 0 0 0; 0.0002488 0 0 0; 0.0003733 0 0 0; 0.0004977 0 0 0; 0.0006221 0 0 0]  x4=[0 0 0 0; 0.0001244 0 0 0; 0.0002488 0 0 0; 0.0003733 0 0 0; 0.0004977 0 0 0; 0.0006221 0 0 0]  x5=0  V1=ones(3,3)  V2=ones(3,3)  I1=ones(3,3)  I2=ones(3,3)  nHarmo=1  Measurements=None
  _CN_93418566_220000_CN_166188874_220000 : powerlib/Elements/Distributed Parameters Line  Phases=3  Frequency=60  Resistance=[0.01273 0.3864]  Inductance="[0.9337e-3  4.1264e-3]"  Capacitance=[12.74e-9 7.751e-9]  Length=6.7474  x1=[0 0 0 0; 0.0001244 0 0 0; 0.0002488 0 0 0; 0.0003733 0 0 0; 0.0004977 0 0 0; 0.0006221 0 0 0]  x2=[0 0 0 0; 0.0001244 0 0 0; 0.0002488 0 0 0; 0.0003733 0 0 0; 0.0004977 0 0 0; 0.0006221 0 0 0]  x3=[0 0 0 0; 0.0001244 0 0 0; 0.0002488 0 0 0; 0.0003733 0 0 0; 0.0004977 0 0 0; 0.0006221 0 0 0]  x4=[0 0 0 0; 0.0001244 0 0 0; 0.0002488 0 0 0; 0.0003733 0 0 0; 0.0004977 0 0 0; 0.0006221 0 0 0]  x5=0  V1=ones(3,3)  V2=ones(3,3)  I1=ones(3,3)  I2=ones(3,3)  nHarmo=1  Measurements=None
  _CN_94087563_220000_CN_130506016_220000 : powerlib/Elements/Distributed Parameters Line  Phases=3  Frequency=60  Resistance=[0.01273 0.3864]  Inductance="[0.9337e-3  4.1264e-3]"  Capacitance=[12.74e-9 7.751e-9]  Length=9.0375  x1=[0 0 0 0; 0.0001244 0 0 0; 0.0002488 0 0 0; 0.0003733 0 0 0; 0.0004977 0 0 0; 0.0006221 0 0 0]  x2=[0 0 0 0; 0.0001244 0 0 0; 0.0002488 0 0 0; 0.0003733 0 0 0; 0.0004977 0 0 0; 0.0006221 0 0 0]  x3=[0 0 0 0; 0.0001244 0 0 0; 0.0002488 0 0 0; 0.0003733 0 0 0; 0.0004977 0 0 0; 0.0006221 0 0 0]  x4=[0 0 0 0; 0.0001244 0 0 0; 0.0002488 0 0 0; 0.0003733 0 0 0; 0.0004977 0 0 0; 0.0006221 0 0 0]  x5=0  V1=ones(3,3)  V2=ones(3,3)  I1=ones(3,3)  I2=ones(3,3)  nHarmo=1  Measurements=None
  _CN_96842811_110000_CN_254457038_110000 : powerlib/Elements/Distributed Parameters Line  Phases=3  Frequency=60  Resistance=[0.01273 0.3864]  Inductance="[0.9337e-3  4.1264e-3]"  Capacitance=[12.74e-9 7.751e-9]  Length=26.1776  x1=[0 0 0 0; 0.0001244 0 0 0; 0.0002488 0 0 0; 0.0003733 0 0 0; 0.0004977 0 0 0; 0.0006221 0 0 0]  x2=[0 0 0 0; 0.0001244 0 0 0; 0.0002488 0 0 0; 0.0003733 0 0 0; 0.0004977 0 0 0; 0.0006221 0 0 0]  x3=[0 0 0 0; 0.0001244 0 0 0; 0.0002488 0 0 0; 0.0003733 0 0 0; 0.0004977 0 0 0; 0.0006221 0 0 0]  x4=[0 0 0 0; 0.0001244 0 0 0; 0.0002488 0 0 0; 0.0003733 0 0 0; 0.0004977 0 0 0; 0.0006221 0 0 0]  x5=0  V1=ones(3,3)  V2=ones(3,3)  I1=ones(3,3)  I2=ones(3,3)  nHarmo=1  Measurements=None
  _CN_96842811_110000_CN_351136526_110000 : powerlib/Elements/Distributed Parameters Line  Phases=3  Frequency=60  Resistance=[0.01273 0.3864]  Inductance="[0.9337e-3  4.1264e-3]"  Capacitance=[12.74e-9 7.751e-9]  Length=9.6129  x1=[0 0 0 0; 0.0001244 0 0 0; 0.0002488 0 0 0; 0.0003733 0 0 0; 0.0004977 0 0 0; 0.0006221 0 0 0]  x2=[0 0 0 0; 0.0001244 0 0 0; 0.0002488 0 0 0; 0.0003733 0 0 0; 0.0004977 0 0 0; 0.0006221 0 0 0]  x3=[0 0 0 0; 0.0001244 0 0 0; 0.0002488 0 0 0; 0.0003733 0 0 0; 0.0004977 0 0 0; 0.0006221 0 0 0]  x4=[0 0 0 0; 0.0001244 0 0 0; 0.0002488 0 0 0; 0.0003733 0 0 0; 0.0004977 0 0 0; 0.0006221 0 0 0]  x5=0  V1=ones(3,3)  V2=ones(3,3)  I1=ones(3,3)  I2=ones(3,3)  nHarmo=1  Measurements=None
  _CN_96989708_220000_CN_81131204_220000 : powerlib/Elements/Distributed Parameters Line  Phases=3  Frequency=60  Resistance=[0.01273 0.3864]  Inductance="[0.9337e-3  4.1264e-3]"  Capacitance=[12.74e-9 7.751e-9]  Length=24.4157  x1=[0 0 0 0; 0.0001244 0 0 0; 0.0002488 0 0 0; 0.0003733 0 0 0; 0.0004977 0 0 0; 0.0006221 0 0 0]  x2=[0 0 0 0; 0.0001244 0 0 0; 0.0002488 0 0 0; 0.0003733 0 0 0; 0.0004977 0 0 0; 0.0006221 0 0 0]  x3=[0 0 0 0; 0.0001244 0 0 0; 0.0002488 0 0 0; 0.0003733 0 0 0; 0.0004977 0 0 0; 0.0006221 0 0 0]  x4=[0 0 0 0; 0.0001244 0 0 0; 0.0002488 0 0 0; 0.0003733 0 0 0; 0.0004977 0 0 0; 0.0006221 0 0 0]  x5=0  V1=ones(3,3)  V2=ones(3,3)  I1=ones(3,3)  I2=ones(3,3)  nHarmo=1  Measurements=None
  _CN_96989715_110000_CN_93260139_110000 : powerlib/Elements/Distributed Parameters Line  Phases=3  Frequency=60  Resistance=[0.01273 0.3864]  Inductance="[0.9337e-3  4.1264e-3]"  Capacitance=[12.74e-9 7.751e-9]  Length=8.7483  x1=[0 0 0 0; 0.0001244 0 0 0; 0.0002488 0 0 0; 0.0003733 0 0 0; 0.0004977 0 0 0; 0.0006221 0 0 0]  x2=[0 0 0 0; 0.0001244 0 0 0; 0.0002488 0 0 0; 0.0003733 0 0 0; 0.0004977 0 0 0; 0.0006221 0 0 0]  x3=[0 0 0 0; 0.0001244 0 0 0; 0.0002488 0 0 0; 0.0003733 0 0 0; 0.0004977 0 0 0; 0.0006221 0 0 0]  x4=[0 0 0 0; 0.0001244 0 0 0; 0.0002488 0 0 0; 0.0003733 0 0 0; 0.0004977 0 0 0; 0.0006221 0 0 0]  x5=0  V1=ones(3,3)  V2=ones(3,3)  I1=ones(3,3)  I2=ones(3,3)  nHarmo=1  Measurements=None
  _CN_97947939_110000_CN_176374151_110000 : powerlib/Elements/Distributed Parameters Line  Phases=3  Frequency=60  Resistance=[0.01273 0.3864]  Inductance="[0.9337e-3  4.1264e-3]"  Capacitance=[12.74e-9 7.751e-9]  Length=9.2276  x1=[0 0 0 0; 0.0001244 0 0 0; 0.0002488 0 0 0; 0.0003733 0 0 0; 0.0004977 0 0 0; 0.0006221 0 0 0]  x2=[0 0 0 0; 0.0001244 0 0 0; 0.0002488 0 0 0; 0.0003733 0 0 0; 0.0004977 0 0 0; 0.0006221 0 0 0]  x3=[0 0 0 0; 0.0001244 0 0 0; 0.0002488 0 0 0; 0.0003733 0 0 0; 0.0004977 0 0 0; 0.0006221 0 0 0]  x4=[0 0 0 0; 0.0001244 0 0 0; 0.0002488 0 0 0; 0.0003733 0 0 0; 0.0004977 0 0 0; 0.0006221 0 0 0]  x5=0  V1=ones(3,3)  V2=ones(3,3)  I1=ones(3,3)  I2=ones(3,3)  nHarmo=1  Measurements=None
  _CN_97947939_110000_CN_38919677_110000 : powerlib/Elements/Distributed Parameters Line  Phases=3  Frequency=60  Resistance=[0.01273 0.3864]  Inductance="[0.9337e-3  4.1264e-3]"  Capacitance=[12.74e-9 7.751e-9]  Length=15.6156  x1=[0 0 0 0; 0.0001244 0 0 0; 0.0002488 0 0 0; 0.0003733 0 0 0; 0.0004977 0 0 0; 0.0006221 0 0 0]  x2=[0 0 0 0; 0.0001244 0 0 0; 0.0002488 0 0 0; 0.0003733 0 0 0; 0.0004977 0 0 0; 0.0006221 0 0 0]  x3=[0 0 0 0; 0.0001244 0 0 0; 0.0002488 0 0 0; 0.0003733 0 0 0; 0.0004977 0 0 0; 0.0006221 0 0 0]  x4=[0 0 0 0; 0.0001244 0 0 0; 0.0002488 0 0 0; 0.0003733 0 0 0; 0.0004977 0 0 0; 0.0006221 0 0 0]  x5=0  V1=ones(3,3)  V2=ones(3,3)  I1=ones(3,3)  I2=ones(3,3)  nHarmo=1  Measurements=None
  _CN_98423617_220000_CN_102963612_220000 : powerlib/Elements/Distributed Parameters Line  Phases=3  Frequency=60  Resistance=[0.01273 0.3864]  Inductance="[0.9337e-3  4.1264e-3]"  Capacitance=[12.74e-9 7.751e-9]  Length=34.3739  x1=[0 0 0 0; 0.0001244 0 0 0; 0.0002488 0 0 0; 0.0003733 0 0 0; 0.0004977 0 0 0; 0.0006221 0 0 0]  x2=[0 0 0 0; 0.0001244 0 0 0; 0.0002488 0 0 0; 0.0003733 0 0 0; 0.0004977 0 0 0; 0.0006221 0 0 0]  x3=[0 0 0 0; 0.0001244 0 0 0; 0.0002488 0 0 0; 0.0003733 0 0 0; 0.0004977 0 0 0; 0.0006221 0 0 0]  x4=[0 0 0 0; 0.0001244 0 0 0; 0.0002488 0 0 0; 0.0003733 0 0 0; 0.0004977 0 0 0; 0.0006221 0 0 0]  x5=0  V1=ones(3,3)  V2=ones(3,3)  I1=ones(3,3)  I2=ones(3,3)  nHarmo=1  Measurements=None
  _CN_98423617_220000_CN_106808187_220000 : powerlib/Elements/Distributed Parameters Line  Phases=3  Frequency=60  Resistance=[0.01273 0.3864]  Inductance="[0.9337e-3  4.1264e-3]"  Capacitance=[12.74e-9 7.751e-9]  Length=8.0978  x1=[0 0 0 0; 0.0001244 0 0 0; 0.0002488 0 0 0; 0.0003733 0 0 0; 0.0004977 0 0 0; 0.0006221 0 0 0]  x2=[0 0 0 0; 0.0001244 0 0 0; 0.0002488 0 0 0; 0.0003733 0 0 0; 0.0004977 0 0 0; 0.0006221 0 0 0]  x3=[0 0 0 0; 0.0001244 0 0 0; 0.0002488 0 0 0; 0.0003733 0 0 0; 0.0004977 0 0 0; 0.0006221 0 0 0]  x4=[0 0 0 0; 0.0001244 0 0 0; 0.0002488 0 0 0; 0.0003733 0 0 0; 0.0004977 0 0 0; 0.0006221 0 0 0]  x5=0  V1=ones(3,3)  V2=ones(3,3)  I1=ones(3,3)  I2=ones(3,3)  nHarmo=1  Measurements=None
  _CN_98423617_220000_CN_109226934_220000 : powerlib/Elements/Distributed Parameters Line  Phases=3  Frequency=60  Resistance=[0.01273 0.3864]  Inductance="[0.9337e-3  4.1264e-3]"  Capacitance=[12.74e-9 7.751e-9]  Length=36.5831  x1=[0 0 0 0; 0.0001244 0 0 0; 0.0002488 0 0 0; 0.0003733 0 0 0; 0.0004977 0 0 0; 0.0006221 0 0 0]  x2=[0 0 0 0; 0.0001244 0 0 0; 0.0002488 0 0 0; 0.0003733 0 0 0; 0.0004977 0 0 0; 0.0006221 0 0 0]  x3=[0 0 0 0; 0.0001244 0 0 0; 0.0002488 0 0 0; 0.0003733 0 0 0; 0.0004977 0 0 0; 0.0006221 0 0 0]  x4=[0 0 0 0; 0.0001244 0 0 0; 0.0002488 0 0 0; 0.0003733 0 0 0; 0.0004977 0 0 0; 0.0006221 0 0 0]  x5=0  V1=ones(3,3)  V2=ones(3,3)  I1=ones(3,3)  I2=ones(3,3)  nHarmo=1  Measurements=None
  _CN_98423617_220000_CN_166188874_220000 : powerlib/Elements/Distributed Parameters Line  Phases=3  Frequency=60  Resistance=[0.01273 0.3864]  Inductance="[0.9337e-3  4.1264e-3]"  Capacitance=[12.74e-9 7.751e-9]  Length=97.5457  x1=[0 0 0 0; 0.0001244 0 0 0; 0.0002488 0 0 0; 0.0003733 0 0 0; 0.0004977 0 0 0; 0.0006221 0 0 0]  x2=[0 0 0 0; 0.0001244 0 0 0; 0.0002488 0 0 0; 0.0003733 0 0 0; 0.0004977 0 0 0; 0.0006221 0 0 0]  x3=[0 0 0 0; 0.0001244 0 0 0; 0.0002488 0 0 0; 0.0003733 0 0 0; 0.0004977 0 0 0; 0.0006221 0 0 0]  x4=[0 0 0 0; 0.0001244 0 0 0; 0.0002488 0 0 0; 0.0003733 0 0 0; 0.0004977 0 0 0; 0.0006221 0 0 0]  x5=0  V1=ones(3,3)  V2=ones(3,3)  I1=ones(3,3)  I2=ones(3,3)  nHarmo=1  Measurements=None
  _CN_98423617_220000_CN_86338059_220000 : powerlib/Elements/Distributed Parameters Line  Phases=3  Frequency=60  Resistance=[0.01273 0.3864]  Inductance="[0.9337e-3  4.1264e-3]"  Capacitance=[12.74e-9 7.751e-9]  Length=15.7685  x1=[0 0 0 0; 0.0001244 0 0 0; 0.0002488 0 0 0; 0.0003733 0 0 0; 0.0004977 0 0 0; 0.0006221 0 0 0]  x2=[0 0 0 0; 0.0001244 0 0 0; 0.0002488 0 0 0; 0.0003733 0 0 0; 0.0004977 0 0 0; 0.0006221 0 0 0]  x3=[0 0 0 0; 0.0001244 0 0 0; 0.0002488 0 0 0; 0.0003733 0 0 0; 0.0004977 0 0 0; 0.0006221 0 0 0]  x4=[0 0 0 0; 0.0001244 0 0 0; 0.0002488 0 0 0; 0.0003733 0 0 0; 0.0004977 0 0 0; 0.0006221 0 0 0]  x5=0  V1=ones(3,3)  V2=ones(3,3)  I1=ones(3,3)  I2=ones(3,3)  nHarmo=1  Measurements=None
  _CN_98423617_500000_CN_109226934_220000 : powerlib/Elements/Distributed Parameters Line  Phases=3  Frequency=60  Resistance=[0.01273 0.3864]  Inductance="[0.9337e-3  4.1264e-3]"  Capacitance=[12.74e-9 7.751e-9]  Length=57.3988  x1=[0 0 0 0; 0.0001244 0 0 0; 0.0002488 0 0 0; 0.0003733 0 0 0; 0.0004977 0 0 0; 0.0006221 0 0 0]  x2=[0 0 0 0; 0.0001244 0 0 0; 0.0002488 0 0 0; 0.0003733 0 0 0; 0.0004977 0 0 0; 0.0006221 0 0 0]  x3=[0 0 0 0; 0.0001244 0 0 0; 0.0002488 0 0 0; 0.0003733 0 0 0; 0.0004977 0 0 0; 0.0006221 0 0 0]  x4=[0 0 0 0; 0.0001244 0 0 0; 0.0002488 0 0 0; 0.0003733 0 0 0; 0.0004977 0 0 0; 0.0006221 0 0 0]  x5=0  V1=ones(3,3)  V2=ones(3,3)  I1=ones(3,3)  I2=ones(3,3)  nHarmo=1  Measurements=None
  _CN_98423617_500000_CN_117237579_500000 : powerlib/Elements/Distributed Parameters Line  Phases=3  Frequency=60  Resistance=[0.01273 0.3864]  Inductance="[0.9337e-3  4.1264e-3]"  Capacitance=[12.74e-9 7.751e-9]  Length=55.2316  x1=[0 0 0 0; 0.0001244 0 0 0; 0.0002488 0 0 0; 0.0003733 0 0 0; 0.0004977 0 0 0; 0.0006221 0 0 0]  x2=[0 0 0 0; 0.0001244 0 0 0; 0.0002488 0 0 0; 0.0003733 0 0 0; 0.0004977 0 0 0; 0.0006221 0 0 0]  x3=[0 0 0 0; 0.0001244 0 0 0; 0.0002488 0 0 0; 0.0003733 0 0 0; 0.0004977 0 0 0; 0.0006221 0 0 0]  x4=[0 0 0 0; 0.0001244 0 0 0; 0.0002488 0 0 0; 0.0003733 0 0 0; 0.0004977 0 0 0; 0.0006221 0 0 0]  x5=0  V1=ones(3,3)  V2=ones(3,3)  I1=ones(3,3)  I2=ones(3,3)  nHarmo=1  Measurements=None
  _CN_99190583_500000_CN_219112646_500000 : powerlib/Elements/Distributed Parameters Line  Phases=3  Frequency=60  Resistance=[0.01273 0.3864]  Inductance="[0.9337e-3  4.1264e-3]"  Capacitance=[12.74e-9 7.751e-9]  Length=15.8707  x1=[0 0 0 0; 0.0001244 0 0 0; 0.0002488 0 0 0; 0.0003733 0 0 0; 0.0004977 0 0 0; 0.0006221 0 0 0]  x2=[0 0 0 0; 0.0001244 0 0 0; 0.0002488 0 0 0; 0.0003733 0 0 0; 0.0004977 0 0 0; 0.0006221 0 0 0]  x3=[0 0 0 0; 0.0001244 0 0 0; 0.0002488 0 0 0; 0.0003733 0 0 0; 0.0004977 0 0 0; 0.0006221 0 0 0]  x4=[0 0 0 0; 0.0001244 0 0 0; 0.0002488 0 0 0; 0.0003733 0 0 0; 0.0004977 0 0 0; 0.0006221 0 0 0]  x5=0  V1=ones(3,3)  V2=ones(3,3)  I1=ones(3,3)  I2=ones(3,3)  nHarmo=1  Measurements=None
  _CN_99731541_110000_CN_101747976_110000 : powerlib/Elements/Distributed Parameters Line  Phases=3  Frequency=60  Resistance=[0.01273 0.3864]  Inductance="[0.9337e-3  4.1264e-3]"  Capacitance=[12.74e-9 7.751e-9]  Length=5.2575  x1=[0 0 0 0; 0.0001244 0 0 0; 0.0002488 0 0 0; 0.0003733 0 0 0; 0.0004977 0 0 0; 0.0006221 0 0 0]  x2=[0 0 0 0; 0.0001244 0 0 0; 0.0002488 0 0 0; 0.0003733 0 0 0; 0.0004977 0 0 0; 0.0006221 0 0 0]  x3=[0 0 0 0; 0.0001244 0 0 0; 0.0002488 0 0 0; 0.0003733 0 0 0; 0.0004977 0 0 0; 0.0006221 0 0 0]  x4=[0 0 0 0; 0.0001244 0 0 0; 0.0002488 0 0 0; 0.0003733 0 0 0; 0.0004977 0 0 0; 0.0006221 0 0 0]  x5=0  V1=ones(3,3)  V2=ones(3,3)  I1=ones(3,3)  I2=ones(3,3)  nHarmo=1  Measurements=None
  _CN_99875927_110000_CN_101594027_110000 : powerlib/Elements/Distributed Parameters Line  Phases=3  Frequency=60  Resistance=[0.01273 0.3864]  Inductance="[0.9337e-3  4.1264e-3]"  Capacitance=[12.74e-9 7.751e-9]  Length=2.0958  x1=[0 0 0 0; 0.0001244 0 0 0; 0.0002488 0 0 0; 0.0003733 0 0 0; 0.0004977 0 0 0; 0.0006221 0 0 0]  x2=[0 0 0 0; 0.0001244 0 0 0; 0.0002488 0 0 0; 0.0003733 0 0 0; 0.0004977 0 0 0; 0.0006221 0 0 0]  x3=[0 0 0 0; 0.0001244 0 0 0; 0.0002488 0 0 0; 0.0003733 0 0 0; 0.0004977 0 0 0; 0.0006221 0 0 0]  x4=[0 0 0 0; 0.0001244 0 0 0; 0.0002488 0 0 0; 0.0003733 0 0 0; 0.0004977 0 0 0; 0.0006221 0 0 0]  x5=0  V1=ones(3,3)  V2=ones(3,3)  I1=ones(3,3)  I2=ones(3,3)  nHarmo=1  Measurements=None
  _CN_99875927_110000_CN_99869836_110000 : powerlib/Elements/Distributed Parameters Line  Phases=3  Frequency=60  Resistance=[0.01273 0.3864]  Inductance="[0.9337e-3  4.1264e-3]"  Capacitance=[12.74e-9 7.751e-9]  Length=4.6852  x1=[0 0 0 0; 0.0001244 0 0 0; 0.0002488 0 0 0; 0.0003733 0 0 0; 0.0004977 0 0 0; 0.0006221 0 0 0]  x2=[0 0 0 0; 0.0001244 0 0 0; 0.0002488 0 0 0; 0.0003733 0 0 0; 0.0004977 0 0 0; 0.0006221 0 0 0]  x3=[0 0 0 0; 0.0001244 0 0 0; 0.0002488 0 0 0; 0.0003733 0 0 0; 0.0004977 0 0 0; 0.0006221 0 0 0]  x4=[0 0 0 0; 0.0001244 0 0 0; 0.0002488 0 0 0; 0.0003733 0 0 0; 0.0004977 0 0 0; 0.0006221 0 0 0]  x5=0  V1=ones(3,3)  V2=ones(3,3)  I1=ones(3,3)  I2=ones(3,3)  nHarmo=1  Measurements=None
  bus1 : powerlib/Measurements/Load Flow Bus  LConnTagsString=a  ID=bus1  Vbase=110000  Vref=1  Vangle=0  VLF=1  angleLF=0
      settings: AttributesFormatString=|
      | %<ID>
      | %<Vbase>V
      | %<VLF>pu
      | %<angleLF>deg.
      | %<Name>
  bus10 : powerlib/Measurements/Load Flow Bus  LConnTagsString=a  ID=bus10  Vbase=110000  Vref=1  Vangle=0  VLF=1  angleLF=0
      settings: AttributesFormatString=|
      | %<ID>
      | %<Vbase>V
      | %<VLF>pu
      | %<angleLF>deg.
      | %<Name>
  bus100 : powerlib/Measurements/Load Flow Bus  LConnTagsString=a  ID=bus100  Vbase=110000  Vref=1  Vangle=0  VLF=1  angleLF=0
      settings: AttributesFormatString=|
      | %<ID>
      | %<Vbase>V
      | %<VLF>pu
      | %<angleLF>deg.
      | %<Name>
  bus101 : powerlib/Measurements/Load Flow Bus  LConnTagsString=a  ID=bus101  Vbase=110000  Vref=1  Vangle=0  VLF=1  angleLF=0
      settings: AttributesFormatString=|
      | %<ID>
      | %<Vbase>V
      | %<VLF>pu
      | %<angleLF>deg.
      | %<Name>
  bus102 : powerlib/Measurements/Load Flow Bus  LConnTagsString=a  ID=bus102  Vbase=110000  Vref=1  Vangle=0  VLF=1  angleLF=0
      settings: AttributesFormatString=|
      | %<ID>
      | %<Vbase>V
      | %<VLF>pu
      | %<angleLF>deg.
      | %<Name>
  bus103 : powerlib/Measurements/Load Flow Bus  LConnTagsString=a  ID=bus103  Vbase=110000  Vref=1  Vangle=0  VLF=1  angleLF=0
      settings: AttributesFormatString=|
      | %<ID>
      | %<Vbase>V
      | %<VLF>pu
      | %<angleLF>deg.
      | %<Name>
  bus104 : powerlib/Measurements/Load Flow Bus  LConnTagsString=a  ID=bus104  Vbase=110000  Vref=1  Vangle=0  VLF=1  angleLF=0
      settings: AttributesFormatString=|
      | %<ID>
      | %<Vbase>V
      | %<VLF>pu
      | %<angleLF>deg.
      | %<Name>
  bus105 : powerlib/Measurements/Load Flow Bus  LConnTagsString=a  ID=bus105  Vbase=110000  Vref=1  Vangle=0  VLF=1  angleLF=0
      settings: AttributesFormatString=|
      | %<ID>
      | %<Vbase>V
      | %<VLF>pu
      | %<angleLF>deg.
      | %<Name>
  bus106 : powerlib/Measurements/Load Flow Bus  LConnTagsString=a  ID=bus106  Vbase=110000  Vref=1  Vangle=0  VLF=1  angleLF=0
      settings: AttributesFormatString=|
      | %<ID>
      | %<Vbase>V
      | %<VLF>pu
      | %<angleLF>deg.
      | %<Name>
  bus107 : powerlib/Measurements/Load Flow Bus  LConnTagsString=a  ID=bus107  Vbase=110000  Vref=1  Vangle=0  VLF=1  angleLF=0
      settings: AttributesFormatString=|
      | %<ID>
      | %<Vbase>V
      | %<VLF>pu
      | %<angleLF>deg.
      | %<Name>
  bus108 : powerlib/Measurements/Load Flow Bus  LConnTagsString=a  ID=bus108  Vbase=110000  Vref=1  Vangle=0  VLF=1  angleLF=0
      settings: AttributesFormatString=|
      | %<ID>
      | %<Vbase>V
      | %<VLF>pu
      | %<angleLF>deg.
      | %<Name>
  bus109 : powerlib/Measurements/Load Flow Bus  LConnTagsString=a  ID=bus109  Vbase=110000  Vref=1  Vangle=0  VLF=1  angleLF=0
      settings: AttributesFormatString=|
      | %<ID>
      | %<Vbase>V
      | %<VLF>pu
      | %<angleLF>deg.
      | %<Name>
  bus11 : powerlib/Measurements/Load Flow Bus  LConnTagsString=a  ID=bus11  Vbase=110000  Vref=1  Vangle=0  VLF=1  angleLF=0
      settings: AttributesFormatString=|
      | %<ID>
      | %<Vbase>V
      | %<VLF>pu
      | %<angleLF>deg.
      | %<Name>
  bus110 : powerlib/Measurements/Load Flow Bus  LConnTagsString=a  ID=bus110  Vbase=110000  Vref=1  Vangle=0  VLF=1  angleLF=0
      settings: AttributesFormatString=|
      | %<ID>
      | %<Vbase>V
      | %<VLF>pu
      | %<angleLF>deg.
      | %<Name>
  bus111 : powerlib/Measurements/Load Flow Bus  LConnTagsString=a  ID=bus111  Vbase=110000  Vref=1  Vangle=0  VLF=1  angleLF=0
      settings: AttributesFormatString=|
      | %<ID>
      | %<Vbase>V
      | %<VLF>pu
      | %<angleLF>deg.
      | %<Name>
  bus112 : powerlib/Measurements/Load Flow Bus  LConnTagsString=a  ID=bus112  Vbase=110000  Vref=1  Vangle=0  VLF=1  angleLF=0
      settings: AttributesFormatString=|
      | %<ID>
      | %<Vbase>V
      | %<VLF>pu
      | %<angleLF>deg.
      | %<Name>
  bus113 : powerlib/Measurements/Load Flow Bus  LConnTagsString=a  ID=bus113  Vbase=110000  Vref=1  Vangle=0  VLF=1  angleLF=0
      settings: AttributesFormatString=|
      | %<ID>
      | %<Vbase>V
      | %<VLF>pu
      | %<angleLF>deg.
      | %<Name>
  bus114 : powerlib/Measurements/Load Flow Bus  LConnTagsString=a  ID=bus114  Vbase=110000  Vref=1  Vangle=0  VLF=1  angleLF=0
      settings: AttributesFormatString=|
      | %<ID>
      | %<Vbase>V
      | %<VLF>pu
      | %<angleLF>deg.
      | %<Name>
  bus115 : powerlib/Measurements/Load Flow Bus  LConnTagsString=a  ID=bus115  Vbase=110000  Vref=1  Vangle=0  VLF=1  angleLF=0
      settings: AttributesFormatString=|
      | %<ID>
      | %<Vbase>V
      | %<VLF>pu
      | %<angleLF>deg.
      | %<Name>
  bus116 : powerlib/Measurements/Load Flow Bus  LConnTagsString=a  ID=bus116  Vbase=110000  Vref=1  Vangle=0  VLF=1  angleLF=0
      settings: AttributesFormatString=|
      | %<ID>
      | %<Vbase>V
      | %<VLF>pu
      | %<angleLF>deg.
      | %<Name>
  bus117 : powerlib/Measurements/Load Flow Bus  LConnTagsString=a  ID=bus117  Vbase=110000  Vref=1  Vangle=0  VLF=1  angleLF=0
      settings: AttributesFormatString=|
      | %<ID>
      | %<Vbase>V
      | %<VLF>pu
      | %<angleLF>deg.
      | %<Name>
  bus118 : powerlib/Measurements/Load Flow Bus  LConnTagsString=a  ID=bus118  Vbase=110000  Vref=1  Vangle=0  VLF=1  angleLF=0
      settings: AttributesFormatString=|
      | %<ID>
      | %<Vbase>V
      | %<VLF>pu
      | %<angleLF>deg.
      | %<Name>
  bus119 : powerlib/Measurements/Load Flow Bus  LConnTagsString=a  ID=bus119  Vbase=110000  Vref=1  Vangle=0  VLF=1  angleLF=0
      settings: AttributesFormatString=|
      | %<ID>
      | %<Vbase>V
      | %<VLF>pu
      | %<angleLF>deg.
      | %<Name>
  bus12 : powerlib/Measurements/Load Flow Bus  LConnTagsString=a  ID=bus12  Vbase=110000  Vref=1  Vangle=0  VLF=1  angleLF=0
      settings: AttributesFormatString=|
      | %<ID>
      | %<Vbase>V
      | %<VLF>pu
      | %<angleLF>deg.
      | %<Name>
  bus120 : powerlib/Measurements/Load Flow Bus  LConnTagsString=a  ID=bus120  Vbase=110000  Vref=1  Vangle=0  VLF=1  angleLF=0
      settings: AttributesFormatString=|
      | %<ID>
      | %<Vbase>V
      | %<VLF>pu
      | %<angleLF>deg.
      | %<Name>
  bus121 : powerlib/Measurements/Load Flow Bus  LConnTagsString=a  ID=bus121  Vbase=110000  Vref=1  Vangle=0  VLF=1  angleLF=0
      settings: AttributesFormatString=|
      | %<ID>
      | %<Vbase>V
      | %<VLF>pu
      | %<angleLF>deg.
      | %<Name>
  bus122 : powerlib/Measurements/Load Flow Bus  LConnTagsString=a  ID=bus122  Vbase=110000  Vref=1  Vangle=0  VLF=1  angleLF=0
      settings: AttributesFormatString=|
      | %<ID>
      | %<Vbase>V
      | %<VLF>pu
      | %<angleLF>deg.
      | %<Name>
  bus123 : powerlib/Measurements/Load Flow Bus  LConnTagsString=a  ID=bus123  Vbase=110000  Vref=1  Vangle=0  VLF=1  angleLF=0
      settings: AttributesFormatString=|
      | %<ID>
      | %<Vbase>V
      | %<VLF>pu
      | %<angleLF>deg.
      | %<Name>
  bus124 : powerlib/Measurements/Load Flow Bus  LConnTagsString=a  ID=bus124  Vbase=110000  Vref=1  Vangle=0  VLF=1  angleLF=0
      settings: AttributesFormatString=|
      | %<ID>
      | %<Vbase>V
      | %<VLF>pu
      | %<angleLF>deg.
      | %<Name>
  bus125 : powerlib/Measurements/Load Flow Bus  LConnTagsString=a  ID=bus125  Vbase=110000  Vref=1  Vangle=0  VLF=1  angleLF=0
      settings: AttributesFormatString=|
      | %<ID>
      | %<Vbase>V
      | %<VLF>pu
      | %<angleLF>deg.
      | %<Name>
  bus126 : powerlib/Measurements/Load Flow Bus  LConnTagsString=a  ID=bus126  Vbase=110000  Vref=1  Vangle=0  VLF=1  angleLF=0
      settings: AttributesFormatString=|
      | %<ID>
      | %<Vbase>V
      | %<VLF>pu
      | %<angleLF>deg.
      | %<Name>
  bus127 : powerlib/Measurements/Load Flow Bus  LConnTagsString=a  ID=bus127  Vbase=110000  Vref=1  Vangle=0  VLF=1  angleLF=0
      settings: AttributesFormatString=|
      | %<ID>
      | %<Vbase>V
      | %<VLF>pu
      | %<angleLF>deg.
      | %<Name>
  bus128 : powerlib/Measurements/Load Flow Bus  LConnTagsString=a  ID=bus128  Vbase=110000  Vref=1  Vangle=0  VLF=1  angleLF=0
      settings: AttributesFormatString=|
      | %<ID>
      | %<Vbase>V
      | %<VLF>pu
      | %<angleLF>deg.
      | %<Name>
  bus129 : powerlib/Measurements/Load Flow Bus  LConnTagsString=a  ID=bus129  Vbase=110000  Vref=1  Vangle=0  VLF=1  angleLF=0
      settings: AttributesFormatString=|
      | %<ID>
      | %<Vbase>V
      | %<VLF>pu
      | %<angleLF>deg.
      | %<Name>
  bus13 : powerlib/Measurements/Load Flow Bus  LConnTagsString=a  ID=bus13  Vbase=110000  Vref=1  Vangle=0  VLF=1  angleLF=0
      settings: AttributesFormatString=|
      | %<ID>
      | %<Vbase>V
      | %<VLF>pu
      | %<angleLF>deg.
      | %<Name>
  bus130 : powerlib/Measurements/Load Flow Bus  LConnTagsString=a  ID=bus130  Vbase=110000  Vref=1  Vangle=0  VLF=1  angleLF=0
      settings: AttributesFormatString=|
      | %<ID>
      | %<Vbase>V
      | %<VLF>pu
      | %<angleLF>deg.
      | %<Name>
  bus131 : powerlib/Measurements/Load Flow Bus  LConnTagsString=a  ID=bus131  Vbase=110000  Vref=1  Vangle=0  VLF=1  angleLF=0
      settings: AttributesFormatString=|
      | %<ID>
      | %<Vbase>V
      | %<VLF>pu
      | %<angleLF>deg.
      | %<Name>
  bus132 : powerlib/Measurements/Load Flow Bus  LConnTagsString=a  ID=bus132  Vbase=110000  Vref=1  Vangle=0  VLF=1  angleLF=0
      settings: AttributesFormatString=|
      | %<ID>
      | %<Vbase>V
      | %<VLF>pu
      | %<angleLF>deg.
      | %<Name>
  bus133 : powerlib/Measurements/Load Flow Bus  LConnTagsString=a  ID=bus133  Vbase=110000  Vref=1  Vangle=0  VLF=1  angleLF=0
      settings: AttributesFormatString=|
      | %<ID>
      | %<Vbase>V
      | %<VLF>pu
      | %<angleLF>deg.
      | %<Name>
  bus134 : powerlib/Measurements/Load Flow Bus  LConnTagsString=a  ID=bus134  Vbase=110000  Vref=1  Vangle=0  VLF=1  angleLF=0
      settings: AttributesFormatString=|
      | %<ID>
      | %<Vbase>V
      | %<VLF>pu
      | %<angleLF>deg.
      | %<Name>
  bus135 : powerlib/Measurements/Load Flow Bus  LConnTagsString=a  ID=bus135  Vbase=110000  Vref=1  Vangle=0  VLF=1  angleLF=0
      settings: AttributesFormatString=|
      | %<ID>
      | %<Vbase>V
      | %<VLF>pu
      | %<angleLF>deg.
      | %<Name>
  bus136 : powerlib/Measurements/Load Flow Bus  LConnTagsString=a  ID=bus136  Vbase=110000  Vref=1  Vangle=0  VLF=1  angleLF=0
      settings: AttributesFormatString=|
      | %<ID>
      | %<Vbase>V
      | %<VLF>pu
      | %<angleLF>deg.
      | %<Name>
  bus137 : powerlib/Measurements/Load Flow Bus  LConnTagsString=a  ID=bus137  Vbase=110000  Vref=1  Vangle=0  VLF=1  angleLF=0
      settings: AttributesFormatString=|
      | %<ID>
      | %<Vbase>V
      | %<VLF>pu
      | %<angleLF>deg.
      | %<Name>
  bus138 : powerlib/Measurements/Load Flow Bus  LConnTagsString=a  ID=bus138  Vbase=110000  Vref=1  Vangle=0  VLF=1  angleLF=0
      settings: AttributesFormatString=|
      | %<ID>
      | %<Vbase>V
      | %<VLF>pu
      | %<angleLF>deg.
      | %<Name>
  bus139 : powerlib/Measurements/Load Flow Bus  LConnTagsString=a  ID=bus139  Vbase=110000  Vref=1  Vangle=0  VLF=1  angleLF=0
      settings: AttributesFormatString=|
      | %<ID>
      | %<Vbase>V
      | %<VLF>pu
      | %<angleLF>deg.
      | %<Name>
  bus14 : powerlib/Measurements/Load Flow Bus  LConnTagsString=a  ID=bus14  Vbase=110000  Vref=1  Vangle=0  VLF=1  angleLF=0
      settings: AttributesFormatString=|
      | %<ID>
      | %<Vbase>V
      | %<VLF>pu
      | %<angleLF>deg.
      | %<Name>
  bus140 : powerlib/Measurements/Load Flow Bus  LConnTagsString=a  ID=bus140  Vbase=110000  Vref=1  Vangle=0  VLF=1  angleLF=0
      settings: AttributesFormatString=|
      | %<ID>
      | %<Vbase>V
      | %<VLF>pu
      | %<angleLF>deg.
      | %<Name>
  bus141 : powerlib/Measurements/Load Flow Bus  LConnTagsString=a  ID=bus141  Vbase=110000  Vref=1  Vangle=0  VLF=1  angleLF=0
      settings: AttributesFormatString=|
      | %<ID>
      | %<Vbase>V
      | %<VLF>pu
      | %<angleLF>deg.
      | %<Name>
  bus142 : powerlib/Measurements/Load Flow Bus  LConnTagsString=a  ID=bus142  Vbase=110000  Vref=1  Vangle=0  VLF=1  angleLF=0
      settings: AttributesFormatString=|
      | %<ID>
      | %<Vbase>V
      | %<VLF>pu
      | %<angleLF>deg.
      | %<Name>
  bus143 : powerlib/Measurements/Load Flow Bus  LConnTagsString=a  ID=bus143  Vbase=110000  Vref=1  Vangle=0  VLF=1  angleLF=0
      settings: AttributesFormatString=|
      | %<ID>
      | %<Vbase>V
      | %<VLF>pu
      | %<angleLF>deg.
      | %<Name>
  bus144 : powerlib/Measurements/Load Flow Bus  LConnTagsString=a  ID=bus144  Vbase=110000  Vref=1  Vangle=0  VLF=1  angleLF=0
      settings: AttributesFormatString=|
      | %<ID>
      | %<Vbase>V
      | %<VLF>pu
      | %<angleLF>deg.
      | %<Name>
  bus145 : powerlib/Measurements/Load Flow Bus  LConnTagsString=a  ID=bus145  Vbase=110000  Vref=1  Vangle=0  VLF=1  angleLF=0
      settings: AttributesFormatString=|
      | %<ID>
      | %<Vbase>V
      | %<VLF>pu
      | %<angleLF>deg.
      | %<Name>
  bus146 : powerlib/Measurements/Load Flow Bus  LConnTagsString=a  ID=bus146  Vbase=110000  Vref=1  Vangle=0  VLF=1  angleLF=0
      settings: AttributesFormatString=|
      | %<ID>
      | %<Vbase>V
      | %<VLF>pu
      | %<angleLF>deg.
      | %<Name>
  bus147 : powerlib/Measurements/Load Flow Bus  LConnTagsString=a  ID=bus147  Vbase=110000  Vref=1  Vangle=0  VLF=1  angleLF=0
      settings: AttributesFormatString=|
      | %<ID>
      | %<Vbase>V
      | %<VLF>pu
      | %<angleLF>deg.
      | %<Name>
  bus148 : powerlib/Measurements/Load Flow Bus  LConnTagsString=a  ID=bus148  Vbase=110000  Vref=1  Vangle=0  VLF=1  angleLF=0
      settings: AttributesFormatString=|
      | %<ID>
      | %<Vbase>V
      | %<VLF>pu
      | %<angleLF>deg.
      | %<Name>
  bus149 : powerlib/Measurements/Load Flow Bus  LConnTagsString=a  ID=bus149  Vbase=220000  Vref=1  Vangle=0  VLF=1  angleLF=0
      settings: AttributesFormatString=|
      | %<ID>
      | %<Vbase>V
      | %<VLF>pu
      | %<angleLF>deg.
      | %<Name>
  bus15 : powerlib/Measurements/Load Flow Bus  LConnTagsString=a  ID=bus15  Vbase=110000  Vref=1  Vangle=0  VLF=1  angleLF=0
      settings: AttributesFormatString=|
      | %<ID>
      | %<Vbase>V
      | %<VLF>pu
      | %<angleLF>deg.
      | %<Name>
  bus150 : powerlib/Measurements/Load Flow Bus  LConnTagsString=a  ID=bus150  Vbase=220000  Vref=1  Vangle=0  VLF=1  angleLF=0
      settings: AttributesFormatString=|
      | %<ID>
      | %<Vbase>V
      | %<VLF>pu
      | %<angleLF>deg.
      | %<Name>
  bus151 : powerlib/Measurements/Load Flow Bus  LConnTagsString=a  ID=bus151  Vbase=220000  Vref=1  Vangle=0  VLF=1  angleLF=0
      settings: AttributesFormatString=|
      | %<ID>
      | %<Vbase>V
      | %<VLF>pu
      | %<angleLF>deg.
      | %<Name>
  bus152 : powerlib/Measurements/Load Flow Bus  LConnTagsString=a  ID=bus152  Vbase=220000  Vref=1  Vangle=0  VLF=1  angleLF=0
      settings: AttributesFormatString=|
      | %<ID>
      | %<Vbase>V
      | %<VLF>pu
      | %<angleLF>deg.
      | %<Name>
  bus153 : powerlib/Measurements/Load Flow Bus  LConnTagsString=a  ID=bus153  Vbase=220000  Vref=1  Vangle=0  VLF=1  angleLF=0
      settings: AttributesFormatString=|
      | %<ID>
      | %<Vbase>V
      | %<VLF>pu
      | %<angleLF>deg.
      | %<Name>
  bus154 : powerlib/Measurements/Load Flow Bus  LConnTagsString=a  ID=bus154  Vbase=220000  Vref=1  Vangle=0  VLF=1  angleLF=0
      settings: AttributesFormatString=|
      | %<ID>
      | %<Vbase>V
      | %<VLF>pu
      | %<angleLF>deg.
      | %<Name>
  bus155 : powerlib/Measurements/Load Flow Bus  LConnTagsString=a  ID=bus155  Vbase=220000  Vref=1  Vangle=0  VLF=1  angleLF=0
      settings: AttributesFormatString=|
      | %<ID>
      | %<Vbase>V
      | %<VLF>pu
      | %<angleLF>deg.
      | %<Name>
  bus156 : powerlib/Measurements/Load Flow Bus  LConnTagsString=a  ID=bus156  Vbase=220000  Vref=1  Vangle=0  VLF=1  angleLF=0
      settings: AttributesFormatString=|
      | %<ID>
      | %<Vbase>V
      | %<VLF>pu
      | %<angleLF>deg.
      | %<Name>
  bus157 : powerlib/Measurements/Load Flow Bus  LConnTagsString=a  ID=bus157  Vbase=220000  Vref=1  Vangle=0  VLF=1  angleLF=0
      settings: AttributesFormatString=|
      | %<ID>
      | %<Vbase>V
      | %<VLF>pu
      | %<angleLF>deg.
      | %<Name>
  bus158 : powerlib/Measurements/Load Flow Bus  LConnTagsString=a  ID=bus158  Vbase=220000  Vref=1  Vangle=0  VLF=1  angleLF=0
      settings: AttributesFormatString=|
      | %<ID>
      | %<Vbase>V
      | %<VLF>pu
      | %<angleLF>deg.
      | %<Name>
  bus159 : powerlib/Measurements/Load Flow Bus  LConnTagsString=a  ID=bus159  Vbase=220000  Vref=1  Vangle=0  VLF=1  angleLF=0
      settings: AttributesFormatString=|
      | %<ID>
      | %<Vbase>V
      | %<VLF>pu
      | %<angleLF>deg.
      | %<Name>
  bus16 : powerlib/Measurements/Load Flow Bus  LConnTagsString=a  ID=bus16  Vbase=110000  Vref=1  Vangle=0  VLF=1  angleLF=0
      settings: AttributesFormatString=|
      | %<ID>
      | %<Vbase>V
      | %<VLF>pu
      | %<angleLF>deg.
      | %<Name>
  bus160 : powerlib/Measurements/Load Flow Bus  LConnTagsString=a  ID=bus160  Vbase=220000  Vref=1  Vangle=0  VLF=1  angleLF=0
      settings: AttributesFormatString=|
      | %<ID>
      | %<Vbase>V
      | %<VLF>pu
      | %<angleLF>deg.
      | %<Name>
  bus161 : powerlib/Measurements/Load Flow Bus  LConnTagsString=a  ID=bus161  Vbase=220000  Vref=1  Vangle=0  VLF=1  angleLF=0
      settings: AttributesFormatString=|
      | %<ID>
      | %<Vbase>V
      | %<VLF>pu
      | %<angleLF>deg.
      | %<Name>
  bus162 : powerlib/Measurements/Load Flow Bus  LConnTagsString=a  ID=bus162  Vbase=220000  Vref=1  Vangle=0  VLF=1  angleLF=0
      settings: AttributesFormatString=|
      | %<ID>
      | %<Vbase>V
      | %<VLF>pu
      | %<angleLF>deg.
      | %<Name>
  bus163 : powerlib/Measurements/Load Flow Bus  LConnTagsString=a  ID=bus163  Vbase=220000  Vref=1  Vangle=0  VLF=1  angleLF=0
      settings: AttributesFormatString=|
      | %<ID>
      | %<Vbase>V
      | %<VLF>pu
      | %<angleLF>deg.
      | %<Name>
  bus164 : powerlib/Measurements/Load Flow Bus  LConnTagsString=a  ID=bus164  Vbase=220000  Vref=1  Vangle=0  VLF=1  angleLF=0
      settings: AttributesFormatString=|
      | %<ID>
      | %<Vbase>V
      | %<VLF>pu
      | %<angleLF>deg.
      | %<Name>
  bus165 : powerlib/Measurements/Load Flow Bus  LConnTagsString=a  ID=bus165  Vbase=220000  Vref=1  Vangle=0  VLF=1  angleLF=0
      settings: AttributesFormatString=|
      | %<ID>
      | %<Vbase>V
      | %<VLF>pu
      | %<angleLF>deg.
      | %<Name>
  bus166 : powerlib/Measurements/Load Flow Bus  LConnTagsString=a  ID=bus166  Vbase=220000  Vref=1  Vangle=0  VLF=1  angleLF=0
      settings: AttributesFormatString=|
      | %<ID>
      | %<Vbase>V
      | %<VLF>pu
      | %<angleLF>deg.
      | %<Name>
  bus167 : powerlib/Measurements/Load Flow Bus  LConnTagsString=a  ID=bus167  Vbase=220000  Vref=1  Vangle=0  VLF=1  angleLF=0
      settings: AttributesFormatString=|
      | %<ID>
      | %<Vbase>V
      | %<VLF>pu
      | %<angleLF>deg.
      | %<Name>
  bus168 : powerlib/Measurements/Load Flow Bus  LConnTagsString=a  ID=bus168  Vbase=220000  Vref=1  Vangle=0  VLF=1  angleLF=0
      settings: AttributesFormatString=|
      | %<ID>
      | %<Vbase>V
      | %<VLF>pu
      | %<angleLF>deg.
      | %<Name>
  bus169 : powerlib/Measurements/Load Flow Bus  LConnTagsString=a  ID=bus169  Vbase=220000  Vref=1  Vangle=0  VLF=1  angleLF=0
      settings: AttributesFormatString=|
      | %<ID>
      | %<Vbase>V
      | %<VLF>pu
      | %<angleLF>deg.
      | %<Name>
  bus17 : powerlib/Measurements/Load Flow Bus  LConnTagsString=a  ID=bus17  Vbase=110000  Vref=1  Vangle=0  VLF=1  angleLF=0
      settings: AttributesFormatString=|
      | %<ID>
      | %<Vbase>V
      | %<VLF>pu
      | %<angleLF>deg.
      | %<Name>
  bus170 : powerlib/Measurements/Load Flow Bus  LConnTagsString=a  ID=bus170  Vbase=220000  Vref=1  Vangle=0  VLF=1  angleLF=0
      settings: AttributesFormatString=|
      | %<ID>
      | %<Vbase>V
      | %<VLF>pu
      | %<angleLF>deg.
      | %<Name>
  bus171 : powerlib/Measurements/Load Flow Bus  LConnTagsString=a  ID=bus171  Vbase=220000  Vref=1  Vangle=0  VLF=1  angleLF=0
      settings: AttributesFormatString=|
      | %<ID>
      | %<Vbase>V
      | %<VLF>pu
      | %<angleLF>deg.
      | %<Name>
  bus172 : powerlib/Measurements/Load Flow Bus  LConnTagsString=a  ID=bus172  Vbase=220000  Vref=1  Vangle=0  VLF=1  angleLF=0
      settings: AttributesFormatString=|
      | %<ID>
      | %<Vbase>V
      | %<VLF>pu
      | %<angleLF>deg.
      | %<Name>
  bus173 : powerlib/Measurements/Load Flow Bus  LConnTagsString=a  ID=bus173  Vbase=220000  Vref=1  Vangle=0  VLF=1  angleLF=0
      settings: AttributesFormatString=|
      | %<ID>
      | %<Vbase>V
      | %<VLF>pu
      | %<angleLF>deg.
      | %<Name>
  bus174 : powerlib/Measurements/Load Flow Bus  LConnTagsString=a  ID=bus174  Vbase=220000  Vref=1  Vangle=0  VLF=1  angleLF=0
      settings: AttributesFormatString=|
      | %<ID>
      | %<Vbase>V
      | %<VLF>pu
      | %<angleLF>deg.
      | %<Name>
  bus175 : powerlib/Measurements/Load Flow Bus  LConnTagsString=a  ID=bus175  Vbase=220000  Vref=1  Vangle=0  VLF=1  angleLF=0
      settings: AttributesFormatString=|
      | %<ID>
      | %<Vbase>V
      | %<VLF>pu
      | %<angleLF>deg.
      | %<Name>
  bus176 : powerlib/Measurements/Load Flow Bus  LConnTagsString=a  ID=bus176  Vbase=220000  Vref=1  Vangle=0  VLF=1  angleLF=0
      settings: AttributesFormatString=|
      | %<ID>
      | %<Vbase>V
      | %<VLF>pu
      | %<angleLF>deg.
      | %<Name>
  bus177 : powerlib/Measurements/Load Flow Bus  LConnTagsString=a  ID=bus177  Vbase=220000  Vref=1  Vangle=0  VLF=1  angleLF=0
      settings: AttributesFormatString=|
      | %<ID>
      | %<Vbase>V
      | %<VLF>pu
      | %<angleLF>deg.
      | %<Name>
  bus178 : powerlib/Measurements/Load Flow Bus  LConnTagsString=a  ID=bus178  Vbase=220000  Vref=1  Vangle=0  VLF=1  angleLF=0
      settings: AttributesFormatString=|
      | %<ID>
      | %<Vbase>V
      | %<VLF>pu
      | %<angleLF>deg.
      | %<Name>
  bus179 : powerlib/Measurements/Load Flow Bus  LConnTagsString=a  ID=bus179  Vbase=220000  Vref=1  Vangle=0  VLF=1  angleLF=0
      settings: AttributesFormatString=|
      | %<ID>
      | %<Vbase>V
      | %<VLF>pu
      | %<angleLF>deg.
      | %<Name>
  bus18 : powerlib/Measurements/Load Flow Bus  LConnTagsString=a  ID=bus18  Vbase=110000  Vref=1  Vangle=0  VLF=1  angleLF=0
      settings: AttributesFormatString=|
      | %<ID>
      | %<Vbase>V
      | %<VLF>pu
      | %<angleLF>deg.
      | %<Name>
  bus180 : powerlib/Measurements/Load Flow Bus  LConnTagsString=a  ID=bus180  Vbase=220000  Vref=1  Vangle=0  VLF=1  angleLF=0
      settings: AttributesFormatString=|
      | %<ID>
      | %<Vbase>V
      | %<VLF>pu
      | %<angleLF>deg.
      | %<Name>
  bus181 : powerlib/Measurements/Load Flow Bus  LConnTagsString=a  ID=bus181  Vbase=220000  Vref=1  Vangle=0  VLF=1  angleLF=0
      settings: AttributesFormatString=|
      | %<ID>
      | %<Vbase>V
      | %<VLF>pu
      | %<angleLF>deg.
      | %<Name>
  bus182 : powerlib/Measurements/Load Flow Bus  LConnTagsString=a  ID=bus182  Vbase=500000  Vref=1  Vangle=0  VLF=1  angleLF=0
      settings: AttributesFormatString=|
      | %<ID>
      | %<Vbase>V
      | %<VLF>pu
      | %<angleLF>deg.
      | %<Name>
  bus183 : powerlib/Measurements/Load Flow Bus  LConnTagsString=a  ID=bus183  Vbase=500000  Vref=1  Vangle=0  VLF=1  angleLF=0
      settings: AttributesFormatString=|
      | %<ID>
      | %<Vbase>V
      | %<VLF>pu
      | %<angleLF>deg.
      | %<Name>
  bus184 : powerlib/Measurements/Load Flow Bus  LConnTagsString=a  ID=bus184  Vbase=500000  Vref=1  Vangle=0  VLF=1  angleLF=0
      settings: AttributesFormatString=|
      | %<ID>
      | %<Vbase>V
      | %<VLF>pu
      | %<angleLF>deg.
      | %<Name>
  bus185 : powerlib/Measurements/Load Flow Bus  LConnTagsString=a  ID=bus185  Vbase=500000  Vref=1  Vangle=0  VLF=1  angleLF=0
      settings: AttributesFormatString=|
      | %<ID>
      | %<Vbase>V
      | %<VLF>pu
      | %<angleLF>deg.
      | %<Name>
  bus186 : powerlib/Measurements/Load Flow Bus  LConnTagsString=a  ID=bus186  Vbase=500000  Vref=1  Vangle=0  VLF=1  angleLF=0
      settings: AttributesFormatString=|
      | %<ID>
      | %<Vbase>V
      | %<VLF>pu
      | %<angleLF>deg.
      | %<Name>
  bus187 : powerlib/Measurements/Load Flow Bus  LConnTagsString=a  ID=bus187  Vbase=500000  Vref=1  Vangle=0  VLF=1  angleLF=0
      settings: AttributesFormatString=|
      | %<ID>
      | %<Vbase>V
      | %<VLF>pu
      | %<angleLF>deg.
      | %<Name>
  bus188 : powerlib/Measurements/Load Flow Bus  LConnTagsString=a  ID=bus188  Vbase=500000  Vref=1  Vangle=0  VLF=1  angleLF=0
      settings: AttributesFormatString=|
      | %<ID>
      | %<Vbase>V
      | %<VLF>pu
      | %<angleLF>deg.
      | %<Name>
  bus189 : powerlib/Measurements/Load Flow Bus  LConnTagsString=a  ID=bus189  Vbase=500000  Vref=1  Vangle=0  VLF=1  angleLF=0
      settings: AttributesFormatString=|
      | %<ID>
      | %<Vbase>V
      | %<VLF>pu
      | %<angleLF>deg.
      | %<Name>
  bus19 : powerlib/Measurements/Load Flow Bus  LConnTagsString=a  ID=bus19  Vbase=110000  Vref=1  Vangle=0  VLF=1  angleLF=0
      settings: AttributesFormatString=|
      | %<ID>
      | %<Vbase>V
      | %<VLF>pu
      | %<angleLF>deg.
      | %<Name>
  bus190 : powerlib/Measurements/Load Flow Bus  LConnTagsString=a  ID=bus190  Vbase=500000  Vref=1  Vangle=0  VLF=1  angleLF=0
      settings: AttributesFormatString=|
      | %<ID>
      | %<Vbase>V
      | %<VLF>pu
      | %<angleLF>deg.
      | %<Name>
  bus191 : powerlib/Measurements/Load Flow Bus  LConnTagsString=a  ID=bus191  Vbase=500000  Vref=1  Vangle=0  VLF=1  angleLF=0
      settings: AttributesFormatString=|
      | %<ID>
      | %<Vbase>V
      | %<VLF>pu
      | %<angleLF>deg.
      | %<Name>
  bus192 : powerlib/Measurements/Load Flow Bus  LConnTagsString=a  ID=bus192  Vbase=500000  Vref=1  Vangle=0  VLF=1  angleLF=0
      settings: AttributesFormatString=|
      | %<ID>
      | %<Vbase>V
      | %<VLF>pu
      | %<angleLF>deg.
      | %<Name>
  bus193 : powerlib/Measurements/Load Flow Bus  LConnTagsString=a  ID=bus193  Vbase=500000  Vref=1  Vangle=0  VLF=1  angleLF=0
      settings: AttributesFormatString=|
      | %<ID>
      | %<Vbase>V
      | %<VLF>pu
      | %<angleLF>deg.
      | %<Name>
  bus194 : powerlib/Measurements/Load Flow Bus  LConnTagsString=a  ID=bus194  Vbase=500000  Vref=1  Vangle=0  VLF=1  angleLF=0
      settings: AttributesFormatString=|
      | %<ID>
      | %<Vbase>V
      | %<VLF>pu
      | %<angleLF>deg.
      | %<Name>
  bus195 : powerlib/Measurements/Load Flow Bus  LConnTagsString=a  ID=bus195  Vbase=500000  Vref=1  Vangle=0  VLF=1  angleLF=0
      settings: AttributesFormatString=|
      | %<ID>
      | %<Vbase>V
      | %<VLF>pu
      | %<angleLF>deg.
      | %<Name>
  bus196 : powerlib/Measurements/Load Flow Bus  LConnTagsString=a  ID=bus196  Vbase=500000  Vref=1  Vangle=0  VLF=1  angleLF=0
      settings: AttributesFormatString=|
      | %<ID>
      | %<Vbase>V
      | %<VLF>pu
      | %<angleLF>deg.
      | %<Name>
  bus197 : powerlib/Measurements/Load Flow Bus  LConnTagsString=a  ID=bus197  Vbase=500000  Vref=1  Vangle=0  VLF=1  angleLF=0
      settings: AttributesFormatString=|
      | %<ID>
      | %<Vbase>V
      | %<VLF>pu
      | %<angleLF>deg.
      | %<Name>
  bus198 : powerlib/Measurements/Load Flow Bus  LConnTagsString=a  ID=bus198  Vbase=500000  Vref=1  Vangle=0  VLF=1  angleLF=0
      settings: AttributesFormatString=|
      | %<ID>
      | %<Vbase>V
      | %<VLF>pu
      | %<angleLF>deg.
      | %<Name>
  bus199 : powerlib/Measurements/Load Flow Bus  LConnTagsString=a  ID=bus199  Vbase=500000  Vref=1  Vangle=0  VLF=1  angleLF=0
      settings: AttributesFormatString=|
      | %<ID>
      | %<Vbase>V
      | %<VLF>pu
      | %<angleLF>deg.
      | %<Name>
  bus2 : powerlib/Measurements/Load Flow Bus  LConnTagsString=a  ID=bus2  Vbase=110000  Vref=1  Vangle=0  VLF=1  angleLF=0
      settings: AttributesFormatString=|
      | %<ID>
      | %<Vbase>V
      | %<VLF>pu
      | %<angleLF>deg.
      | %<Name>
  bus20 : powerlib/Measurements/Load Flow Bus  LConnTagsString=a  ID=bus20  Vbase=110000  Vref=1  Vangle=0  VLF=1  angleLF=0
      settings: AttributesFormatString=|
      | %<ID>
      | %<Vbase>V
      | %<VLF>pu
      | %<angleLF>deg.
      | %<Name>
  bus200 : powerlib/Measurements/Load Flow Bus  LConnTagsString=a  ID=bus200  Vbase=500000  Vref=1  Vangle=0  VLF=1  angleLF=0
      settings: AttributesFormatString=|
      | %<ID>
      | %<Vbase>V
      | %<VLF>pu
      | %<angleLF>deg.
      | %<Name>
  bus201 : powerlib/Measurements/Load Flow Bus  LConnTagsString=a  ID=bus201  Vbase=500000  Vref=1  Vangle=0  VLF=1  angleLF=0
      settings: AttributesFormatString=|
      | %<ID>
      | %<Vbase>V
      | %<VLF>pu
      | %<angleLF>deg.
      | %<Name>
  bus202 : powerlib/Measurements/Load Flow Bus  LConnTagsString=a  ID=bus202  Vbase=500000  Vref=1  Vangle=0  VLF=1  angleLF=0
      settings: AttributesFormatString=|
      | %<ID>
      | %<Vbase>V
      | %<VLF>pu
      | %<angleLF>deg.
      | %<Name>
  bus203 : powerlib/Measurements/Load Flow Bus  LConnTagsString=a  ID=bus203  Vbase=110000  Vref=1  Vangle=0  VLF=1  angleLF=0
      settings: AttributesFormatString=|
      | %<ID>
      | %<Vbase>V
      | %<VLF>pu
      | %<angleLF>deg.
      | %<Name>
  bus204 : powerlib/Measurements/Load Flow Bus  LConnTagsString=a  ID=bus204  Vbase=110000  Vref=1  Vangle=0  VLF=1  angleLF=0
      settings: AttributesFormatString=|
      | %<ID>
      | %<Vbase>V
      | %<VLF>pu
      | %<angleLF>deg.
      | %<Name>
  bus205 : powerlib/Measurements/Load Flow Bus  LConnTagsString=a  ID=bus205  Vbase=110000  Vref=1  Vangle=0  VLF=1  angleLF=0
      settings: AttributesFormatString=|
      | %<ID>
      | %<Vbase>V
      | %<VLF>pu
      | %<angleLF>deg.
      | %<Name>
  bus206 : powerlib/Measurements/Load Flow Bus  LConnTagsString=a  ID=bus206  Vbase=110000  Vref=1  Vangle=0  VLF=1  angleLF=0
      settings: AttributesFormatString=|
      | %<ID>
      | %<Vbase>V
      | %<VLF>pu
      | %<angleLF>deg.
      | %<Name>
  bus207 : powerlib/Measurements/Load Flow Bus  LConnTagsString=a  ID=bus207  Vbase=110000  Vref=1  Vangle=0  VLF=1  angleLF=0
      settings: AttributesFormatString=|
      | %<ID>
      | %<Vbase>V
      | %<VLF>pu
      | %<angleLF>deg.
      | %<Name>
  bus208 : powerlib/Measurements/Load Flow Bus  LConnTagsString=a  ID=bus208  Vbase=110000  Vref=1  Vangle=0  VLF=1  angleLF=0
      settings: AttributesFormatString=|
      | %<ID>
      | %<Vbase>V
      | %<VLF>pu
      | %<angleLF>deg.
      | %<Name>
  bus209 : powerlib/Measurements/Load Flow Bus  LConnTagsString=a  ID=bus209  Vbase=110000  Vref=1  Vangle=0  VLF=1  angleLF=0
      settings: AttributesFormatString=|
      | %<ID>
      | %<Vbase>V
      | %<VLF>pu
      | %<angleLF>deg.
      | %<Name>
  bus21 : powerlib/Measurements/Load Flow Bus  LConnTagsString=a  ID=bus21  Vbase=110000  Vref=1  Vangle=0  VLF=1  angleLF=0
      settings: AttributesFormatString=|
      | %<ID>
      | %<Vbase>V
      | %<VLF>pu
      | %<angleLF>deg.
      | %<Name>
  bus210 : powerlib/Measurements/Load Flow Bus  LConnTagsString=a  ID=bus210  Vbase=110000  Vref=1  Vangle=0  VLF=1  angleLF=0
      settings: AttributesFormatString=|
      | %<ID>
      | %<Vbase>V
      | %<VLF>pu
      | %<angleLF>deg.
      | %<Name>
  bus211 : powerlib/Measurements/Load Flow Bus  LConnTagsString=a  ID=bus211  Vbase=110000  Vref=1  Vangle=0  VLF=1  angleLF=0
      settings: AttributesFormatString=|
      | %<ID>
      | %<Vbase>V
      | %<VLF>pu
      | %<angleLF>deg.
      | %<Name>
  bus212 : powerlib/Measurements/Load Flow Bus  LConnTagsString=a  ID=bus212  Vbase=110000  Vref=1  Vangle=0  VLF=1  angleLF=0
      settings: AttributesFormatString=|
      | %<ID>
      | %<Vbase>V
      | %<VLF>pu
      | %<angleLF>deg.
      | %<Name>
  bus213 : powerlib/Measurements/Load Flow Bus  LConnTagsString=a  ID=bus213  Vbase=110000  Vref=1  Vangle=0  VLF=1  angleLF=0
      settings: AttributesFormatString=|
      | %<ID>
      | %<Vbase>V
      | %<VLF>pu
      | %<angleLF>deg.
      | %<Name>
  bus214 : powerlib/Measurements/Load Flow Bus  LConnTagsString=a  ID=bus214  Vbase=110000  Vref=1  Vangle=0  VLF=1  angleLF=0
      settings: AttributesFormatString=|
      | %<ID>
      | %<Vbase>V
      | %<VLF>pu
      | %<angleLF>deg.
      | %<Name>
  bus215 : powerlib/Measurements/Load Flow Bus  LConnTagsString=a  ID=bus215  Vbase=110000  Vref=1  Vangle=0  VLF=1  angleLF=0
      settings: AttributesFormatString=|
      | %<ID>
      | %<Vbase>V
      | %<VLF>pu
      | %<angleLF>deg.
      | %<Name>
  bus216 : powerlib/Measurements/Load Flow Bus  LConnTagsString=a  ID=bus216  Vbase=110000  Vref=1  Vangle=0  VLF=1  angleLF=0
      settings: AttributesFormatString=|
      | %<ID>
      | %<Vbase>V
      | %<VLF>pu
      | %<angleLF>deg.
      | %<Name>
  bus217 : powerlib/Measurements/Load Flow Bus  LConnTagsString=a  ID=bus217  Vbase=110000  Vref=1  Vangle=0  VLF=1  angleLF=0
      settings: AttributesFormatString=|
      | %<ID>
      | %<Vbase>V
      | %<VLF>pu
      | %<angleLF>deg.
      | %<Name>
  bus218 : powerlib/Measurements/Load Flow Bus  LConnTagsString=a  ID=bus218  Vbase=110000  Vref=1  Vangle=0  VLF=1  angleLF=0
      settings: AttributesFormatString=|
      | %<ID>
      | %<Vbase>V
      | %<VLF>pu
      | %<angleLF>deg.
      | %<Name>
  bus219 : powerlib/Measurements/Load Flow Bus  LConnTagsString=a  ID=bus219  Vbase=110000  Vref=1  Vangle=0  VLF=1  angleLF=0
      settings: AttributesFormatString=|
      | %<ID>
      | %<Vbase>V
      | %<VLF>pu
      | %<angleLF>deg.
      | %<Name>
  bus22 : powerlib/Measurements/Load Flow Bus  LConnTagsString=a  ID=bus22  Vbase=110000  Vref=1  Vangle=0  VLF=1  angleLF=0
      settings: AttributesFormatString=|
      | %<ID>
      | %<Vbase>V
      | %<VLF>pu
      | %<angleLF>deg.
      | %<Name>
  bus220 : powerlib/Measurements/Load Flow Bus  LConnTagsString=a  ID=bus220  Vbase=110000  Vref=1  Vangle=0  VLF=1  angleLF=0
      settings: AttributesFormatString=|
      | %<ID>
      | %<Vbase>V
      | %<VLF>pu
      | %<angleLF>deg.
      | %<Name>
  bus221 : powerlib/Measurements/Load Flow Bus  LConnTagsString=a  ID=bus221  Vbase=110000  Vref=1  Vangle=0  VLF=1  angleLF=0
      settings: AttributesFormatString=|
      | %<ID>
      | %<Vbase>V
      | %<VLF>pu
      | %<angleLF>deg.
      | %<Name>
  bus222 : powerlib/Measurements/Load Flow Bus  LConnTagsString=a  ID=bus222  Vbase=110000  Vref=1  Vangle=0  VLF=1  angleLF=0
      settings: AttributesFormatString=|
      | %<ID>
      | %<Vbase>V
      | %<VLF>pu
      | %<angleLF>deg.
      | %<Name>
  bus223 : powerlib/Measurements/Load Flow Bus  LConnTagsString=a  ID=bus223  Vbase=110000  Vref=1  Vangle=0  VLF=1  angleLF=0
      settings: AttributesFormatString=|
      | %<ID>
      | %<Vbase>V
      | %<VLF>pu
      | %<angleLF>deg.
      | %<Name>
  bus224 : powerlib/Measurements/Load Flow Bus  LConnTagsString=a  ID=bus224  Vbase=110000  Vref=1  Vangle=0  VLF=1  angleLF=0
      settings: AttributesFormatString=|
      | %<ID>
      | %<Vbase>V
      | %<VLF>pu
      | %<angleLF>deg.
      | %<Name>
  bus225 : powerlib/Measurements/Load Flow Bus  LConnTagsString=a  ID=bus225  Vbase=110000  Vref=1  Vangle=0  VLF=1  angleLF=0
      settings: AttributesFormatString=|
      | %<ID>
      | %<Vbase>V
      | %<VLF>pu
      | %<angleLF>deg.
      | %<Name>
  bus226 : powerlib/Measurements/Load Flow Bus  LConnTagsString=a  ID=bus226  Vbase=110000  Vref=1  Vangle=0  VLF=1  angleLF=0
      settings: AttributesFormatString=|
      | %<ID>
      | %<Vbase>V
      | %<VLF>pu
      | %<angleLF>deg.
      | %<Name>
  bus227 : powerlib/Measurements/Load Flow Bus  LConnTagsString=a  ID=bus227  Vbase=110000  Vref=1  Vangle=0  VLF=1  angleLF=0
      settings: AttributesFormatString=|
      | %<ID>
      | %<Vbase>V
      | %<VLF>pu
      | %<angleLF>deg.
      | %<Name>
  bus228 : powerlib/Measurements/Load Flow Bus  LConnTagsString=a  ID=bus228  Vbase=110000  Vref=1  Vangle=0  VLF=1  angleLF=0
      settings: AttributesFormatString=|
      | %<ID>
      | %<Vbase>V
      | %<VLF>pu
      | %<angleLF>deg.
      | %<Name>
  bus229 : powerlib/Measurements/Load Flow Bus  LConnTagsString=a  ID=bus229  Vbase=110000  Vref=1  Vangle=0  VLF=1  angleLF=0
      settings: AttributesFormatString=|
      | %<ID>
      | %<Vbase>V
      | %<VLF>pu
      | %<angleLF>deg.
      | %<Name>
  bus23 : powerlib/Measurements/Load Flow Bus  LConnTagsString=a  ID=bus23  Vbase=110000  Vref=1  Vangle=0  VLF=1  angleLF=0
      settings: AttributesFormatString=|
      | %<ID>
      | %<Vbase>V
      | %<VLF>pu
      | %<angleLF>deg.
      | %<Name>
  bus230 : powerlib/Measurements/Load Flow Bus  LConnTagsString=a  ID=bus230  Vbase=110000  Vref=1  Vangle=0  VLF=1  angleLF=0
      settings: AttributesFormatString=|
      | %<ID>
      | %<Vbase>V
      | %<VLF>pu
      | %<angleLF>deg.
      | %<Name>
  bus231 : powerlib/Measurements/Load Flow Bus  LConnTagsString=a  ID=bus231  Vbase=110000  Vref=1  Vangle=0  VLF=1  angleLF=0
      settings: AttributesFormatString=|
      | %<ID>
      | %<Vbase>V
      | %<VLF>pu
      | %<angleLF>deg.
      | %<Name>
  bus232 : powerlib/Measurements/Load Flow Bus  LConnTagsString=a  ID=bus232  Vbase=110000  Vref=1  Vangle=0  VLF=1  angleLF=0
      settings: AttributesFormatString=|
      | %<ID>
      | %<Vbase>V
      | %<VLF>pu
      | %<angleLF>deg.
      | %<Name>
  bus233 : powerlib/Measurements/Load Flow Bus  LConnTagsString=a  ID=bus233  Vbase=110000  Vref=1  Vangle=0  VLF=1  angleLF=0
      settings: AttributesFormatString=|
      | %<ID>
      | %<Vbase>V
      | %<VLF>pu
      | %<angleLF>deg.
      | %<Name>
  bus234 : powerlib/Measurements/Load Flow Bus  LConnTagsString=a  ID=bus234  Vbase=110000  Vref=1  Vangle=0  VLF=1  angleLF=0
      settings: AttributesFormatString=|
      | %<ID>
      | %<Vbase>V
      | %<VLF>pu
      | %<angleLF>deg.
      | %<Name>
  bus235 : powerlib/Measurements/Load Flow Bus  LConnTagsString=a  ID=bus235  Vbase=110000  Vref=1  Vangle=0  VLF=1  angleLF=0
      settings: AttributesFormatString=|
      | %<ID>
      | %<Vbase>V
      | %<VLF>pu
      | %<angleLF>deg.
      | %<Name>
  bus236 : powerlib/Measurements/Load Flow Bus  LConnTagsString=a  ID=bus236  Vbase=110000  Vref=1  Vangle=0  VLF=1  angleLF=0
      settings: AttributesFormatString=|
      | %<ID>
      | %<Vbase>V
      | %<VLF>pu
      | %<angleLF>deg.
      | %<Name>
  bus237 : powerlib/Measurements/Load Flow Bus  LConnTagsString=a  ID=bus237  Vbase=110000  Vref=1  Vangle=0  VLF=1  angleLF=0
      settings: AttributesFormatString=|
      | %<ID>
      | %<Vbase>V
      | %<VLF>pu
      | %<angleLF>deg.
      | %<Name>
  bus238 : powerlib/Measurements/Load Flow Bus  LConnTagsString=a  ID=bus238  Vbase=110000  Vref=1  Vangle=0  VLF=1  angleLF=0
      settings: AttributesFormatString=|
      | %<ID>
      | %<Vbase>V
      | %<VLF>pu
      | %<angleLF>deg.
      | %<Name>
  bus239 : powerlib/Measurements/Load Flow Bus  LConnTagsString=a  ID=bus239  Vbase=110000  Vref=1  Vangle=0  VLF=1  angleLF=0
      settings: AttributesFormatString=|
      | %<ID>
      | %<Vbase>V
      | %<VLF>pu
      | %<angleLF>deg.
      | %<Name>
  bus24 : powerlib/Measurements/Load Flow Bus  LConnTagsString=a  ID=bus24  Vbase=110000  Vref=1  Vangle=0  VLF=1  angleLF=0
      settings: AttributesFormatString=|
      | %<ID>
      | %<Vbase>V
      | %<VLF>pu
      | %<angleLF>deg.
      | %<Name>
  bus240 : powerlib/Measurements/Load Flow Bus  LConnTagsString=a  ID=bus240  Vbase=110000  Vref=1  Vangle=0  VLF=1  angleLF=0
      settings: AttributesFormatString=|
      | %<ID>
      | %<Vbase>V
      | %<VLF>pu
      | %<angleLF>deg.
      | %<Name>
  bus241 : powerlib/Measurements/Load Flow Bus  LConnTagsString=a  ID=bus241  Vbase=110000  Vref=1  Vangle=0  VLF=1  angleLF=0
      settings: AttributesFormatString=|
      | %<ID>
      | %<Vbase>V
      | %<VLF>pu
      | %<angleLF>deg.
      | %<Name>
  bus242 : powerlib/Measurements/Load Flow Bus  LConnTagsString=a  ID=bus242  Vbase=110000  Vref=1  Vangle=0  VLF=1  angleLF=0
      settings: AttributesFormatString=|
      | %<ID>
      | %<Vbase>V
      | %<VLF>pu
      | %<angleLF>deg.
      | %<Name>
  bus243 : powerlib/Measurements/Load Flow Bus  LConnTagsString=a  ID=bus243  Vbase=110000  Vref=1  Vangle=0  VLF=1  angleLF=0
      settings: AttributesFormatString=|
      | %<ID>
      | %<Vbase>V
      | %<VLF>pu
      | %<angleLF>deg.
      | %<Name>
  bus244 : powerlib/Measurements/Load Flow Bus  LConnTagsString=a  ID=bus244  Vbase=110000  Vref=1  Vangle=0  VLF=1  angleLF=0
      settings: AttributesFormatString=|
      | %<ID>
      | %<Vbase>V
      | %<VLF>pu
      | %<angleLF>deg.
      | %<Name>
  bus245 : powerlib/Measurements/Load Flow Bus  LConnTagsString=a  ID=bus245  Vbase=110000  Vref=1  Vangle=0  VLF=1  angleLF=0
      settings: AttributesFormatString=|
      | %<ID>
      | %<Vbase>V
      | %<VLF>pu
      | %<angleLF>deg.
      | %<Name>
  bus246 : powerlib/Measurements/Load Flow Bus  LConnTagsString=a  ID=bus246  Vbase=110000  Vref=1  Vangle=0  VLF=1  angleLF=0
      settings: AttributesFormatString=|
      | %<ID>
      | %<Vbase>V
      | %<VLF>pu
      | %<angleLF>deg.
      | %<Name>
  bus247 : powerlib/Measurements/Load Flow Bus  LConnTagsString=a  ID=bus247  Vbase=110000  Vref=1  Vangle=0  VLF=1  angleLF=0
      settings: AttributesFormatString=|
      | %<ID>
      | %<Vbase>V
      | %<VLF>pu
      | %<angleLF>deg.
      | %<Name>
  bus248 : powerlib/Measurements/Load Flow Bus  LConnTagsString=a  ID=bus248  Vbase=110000  Vref=1  Vangle=0  VLF=1  angleLF=0
      settings: AttributesFormatString=|
      | %<ID>
      | %<Vbase>V
      | %<VLF>pu
      | %<angleLF>deg.
      | %<Name>
  bus249 : powerlib/Measurements/Load Flow Bus  LConnTagsString=a  ID=bus249  Vbase=110000  Vref=1  Vangle=0  VLF=1  angleLF=0
      settings: AttributesFormatString=|
      | %<ID>
      | %<Vbase>V
      | %<VLF>pu
      | %<angleLF>deg.
      | %<Name>
  bus25 : powerlib/Measurements/Load Flow Bus  LConnTagsString=a  ID=bus25  Vbase=110000  Vref=1  Vangle=0  VLF=1  angleLF=0
      settings: AttributesFormatString=|
      | %<ID>
      | %<Vbase>V
      | %<VLF>pu
      | %<angleLF>deg.
      | %<Name>
  bus250 : powerlib/Measurements/Load Flow Bus  LConnTagsString=a  ID=bus250  Vbase=110000  Vref=1  Vangle=0  VLF=1  angleLF=0
      settings: AttributesFormatString=|
      | %<ID>
      | %<Vbase>V
      | %<VLF>pu
      | %<angleLF>deg.
      | %<Name>
  bus251 : powerlib/Measurements/Load Flow Bus  LConnTagsString=a  ID=bus251  Vbase=110000  Vref=1  Vangle=0  VLF=1  angleLF=0
      settings: AttributesFormatString=|
      | %<ID>
      | %<Vbase>V
      | %<VLF>pu
      | %<angleLF>deg.
      | %<Name>
  bus252 : powerlib/Measurements/Load Flow Bus  LConnTagsString=a  ID=bus252  Vbase=110000  Vref=1  Vangle=0  VLF=1  angleLF=0
      settings: AttributesFormatString=|
      | %<ID>
      | %<Vbase>V
      | %<VLF>pu
      | %<angleLF>deg.
      | %<Name>
  bus253 : powerlib/Measurements/Load Flow Bus  LConnTagsString=a  ID=bus253  Vbase=110000  Vref=1  Vangle=0  VLF=1  angleLF=0
      settings: AttributesFormatString=|
      | %<ID>
      | %<Vbase>V
      | %<VLF>pu
      | %<angleLF>deg.
      | %<Name>
  bus254 : powerlib/Measurements/Load Flow Bus  LConnTagsString=a  ID=bus254  Vbase=110000  Vref=1  Vangle=0  VLF=1  angleLF=0
      settings: AttributesFormatString=|
      | %<ID>
      | %<Vbase>V
      | %<VLF>pu
      | %<angleLF>deg.
      | %<Name>
  bus255 : powerlib/Measurements/Load Flow Bus  LConnTagsString=a  ID=bus255  Vbase=110000  Vref=1  Vangle=0  VLF=1  angleLF=0
      settings: AttributesFormatString=|
      | %<ID>
      | %<Vbase>V
      | %<VLF>pu
      | %<angleLF>deg.
      | %<Name>
  bus256 : powerlib/Measurements/Load Flow Bus  LConnTagsString=a  ID=bus256  Vbase=110000  Vref=1  Vangle=0  VLF=1  angleLF=0
      settings: AttributesFormatString=|
      | %<ID>
      | %<Vbase>V
      | %<VLF>pu
      | %<angleLF>deg.
      | %<Name>
  bus257 : powerlib/Measurements/Load Flow Bus  LConnTagsString=a  ID=bus257  Vbase=110000  Vref=1  Vangle=0  VLF=1  angleLF=0
      settings: AttributesFormatString=|
      | %<ID>
      | %<Vbase>V
      | %<VLF>pu
      | %<angleLF>deg.
      | %<Name>
  bus258 : powerlib/Measurements/Load Flow Bus  LConnTagsString=a  ID=bus258  Vbase=110000  Vref=1  Vangle=0  VLF=1  angleLF=0
      settings: AttributesFormatString=|
      | %<ID>
      | %<Vbase>V
      | %<VLF>pu
      | %<angleLF>deg.
      | %<Name>
  bus259 : powerlib/Measurements/Load Flow Bus  LConnTagsString=a  ID=bus259  Vbase=110000  Vref=1  Vangle=0  VLF=1  angleLF=0
      settings: AttributesFormatString=|
      | %<ID>
      | %<Vbase>V
      | %<VLF>pu
      | %<angleLF>deg.
      | %<Name>
  bus26 : powerlib/Measurements/Load Flow Bus  LConnTagsString=a  ID=bus26  Vbase=110000  Vref=1  Vangle=0  VLF=1  angleLF=0
      settings: AttributesFormatString=|
      | %<ID>
      | %<Vbase>V
      | %<VLF>pu
      | %<angleLF>deg.
      | %<Name>
  bus260 : powerlib/Measurements/Load Flow Bus  LConnTagsString=a  ID=bus260  Vbase=110000  Vref=1  Vangle=0  VLF=1  angleLF=0
      settings: AttributesFormatString=|
      | %<ID>
      | %<Vbase>V
      | %<VLF>pu
      | %<angleLF>deg.
      | %<Name>
  bus261 : powerlib/Measurements/Load Flow Bus  LConnTagsString=a  ID=bus261  Vbase=110000  Vref=1  Vangle=0  VLF=1  angleLF=0
      settings: AttributesFormatString=|
      | %<ID>
      | %<Vbase>V
      | %<VLF>pu
      | %<angleLF>deg.
      | %<Name>
  bus262 : powerlib/Measurements/Load Flow Bus  LConnTagsString=a  ID=bus262  Vbase=110000  Vref=1  Vangle=0  VLF=1  angleLF=0
      settings: AttributesFormatString=|
      | %<ID>
      | %<Vbase>V
      | %<VLF>pu
      | %<angleLF>deg.
      | %<Name>
  bus263 : powerlib/Measurements/Load Flow Bus  LConnTagsString=a  ID=bus263  Vbase=110000  Vref=1  Vangle=0  VLF=1  angleLF=0
      settings: AttributesFormatString=|
      | %<ID>
      | %<Vbase>V
      | %<VLF>pu
      | %<angleLF>deg.
      | %<Name>
  bus264 : powerlib/Measurements/Load Flow Bus  LConnTagsString=a  ID=bus264  Vbase=110000  Vref=1  Vangle=0  VLF=1  angleLF=0
      settings: AttributesFormatString=|
      | %<ID>
      | %<Vbase>V
      | %<VLF>pu
      | %<angleLF>deg.
      | %<Name>
  bus265 : powerlib/Measurements/Load Flow Bus  LConnTagsString=a  ID=bus265  Vbase=110000  Vref=1  Vangle=0  VLF=1  angleLF=0
      settings: AttributesFormatString=|
      | %<ID>
      | %<Vbase>V
      | %<VLF>pu
      | %<angleLF>deg.
      | %<Name>
  bus266 : powerlib/Measurements/Load Flow Bus  LConnTagsString=a  ID=bus266  Vbase=110000  Vref=1  Vangle=0  VLF=1  angleLF=0
      settings: AttributesFormatString=|
      | %<ID>
      | %<Vbase>V
      | %<VLF>pu
      | %<angleLF>deg.
      | %<Name>
  bus267 : powerlib/Measurements/Load Flow Bus  LConnTagsString=a  ID=bus267  Vbase=110000  Vref=1  Vangle=0  VLF=1  angleLF=0
      settings: AttributesFormatString=|
      | %<ID>
      | %<Vbase>V
      | %<VLF>pu
      | %<angleLF>deg.
      | %<Name>
  bus268 : powerlib/Measurements/Load Flow Bus  LConnTagsString=a  ID=bus268  Vbase=110000  Vref=1  Vangle=0  VLF=1  angleLF=0
      settings: AttributesFormatString=|
      | %<ID>
      | %<Vbase>V
      | %<VLF>pu
      | %<angleLF>deg.
      | %<Name>
  bus269 : powerlib/Measurements/Load Flow Bus  LConnTagsString=a  ID=bus269  Vbase=110000  Vref=1  Vangle=0  VLF=1  angleLF=0
      settings: AttributesFormatString=|
      | %<ID>
      | %<Vbase>V
      | %<VLF>pu
      | %<angleLF>deg.
      | %<Name>
  bus27 : powerlib/Measurements/Load Flow Bus  LConnTagsString=a  ID=bus27  Vbase=110000  Vref=1  Vangle=0  VLF=1  angleLF=0
      settings: AttributesFormatString=|
      | %<ID>
      | %<Vbase>V
      | %<VLF>pu
      | %<angleLF>deg.
      | %<Name>
  bus270 : powerlib/Measurements/Load Flow Bus  LConnTagsString=a  ID=bus270  Vbase=110000  Vref=1  Vangle=0  VLF=1  angleLF=0
      settings: AttributesFormatString=|
      | %<ID>
      | %<Vbase>V
      | %<VLF>pu
      | %<angleLF>deg.
      | %<Name>
  bus271 : powerlib/Measurements/Load Flow Bus  LConnTagsString=a  ID=bus271  Vbase=110000  Vref=1  Vangle=0  VLF=1  angleLF=0
      settings: AttributesFormatString=|
      | %<ID>
      | %<Vbase>V
      | %<VLF>pu
      | %<angleLF>deg.
      | %<Name>
  bus272 : powerlib/Measurements/Load Flow Bus  LConnTagsString=a  ID=bus272  Vbase=110000  Vref=1  Vangle=0  VLF=1  angleLF=0
      settings: AttributesFormatString=|
      | %<ID>
      | %<Vbase>V
      | %<VLF>pu
      | %<angleLF>deg.
      | %<Name>
  bus273 : powerlib/Measurements/Load Flow Bus  LConnTagsString=a  ID=bus273  Vbase=110000  Vref=1  Vangle=0  VLF=1  angleLF=0
      settings: AttributesFormatString=|
      | %<ID>
      | %<Vbase>V
      | %<VLF>pu
      | %<angleLF>deg.
      | %<Name>
  bus274 : powerlib/Measurements/Load Flow Bus  LConnTagsString=a  ID=bus274  Vbase=110000  Vref=1  Vangle=0  VLF=1  angleLF=0
      settings: AttributesFormatString=|
      | %<ID>
      | %<Vbase>V
      | %<VLF>pu
      | %<angleLF>deg.
      | %<Name>
  bus275 : powerlib/Measurements/Load Flow Bus  LConnTagsString=a  ID=bus275  Vbase=110000  Vref=1  Vangle=0  VLF=1  angleLF=0
      settings: AttributesFormatString=|
      | %<ID>
      | %<Vbase>V
      | %<VLF>pu
      | %<angleLF>deg.
      | %<Name>
  bus276 : powerlib/Measurements/Load Flow Bus  LConnTagsString=a  ID=bus276  Vbase=110000  Vref=1  Vangle=0  VLF=1  angleLF=0
      settings: AttributesFormatString=|
      | %<ID>
      | %<Vbase>V
      | %<VLF>pu
      | %<angleLF>deg.
      | %<Name>
  bus277 : powerlib/Measurements/Load Flow Bus  LConnTagsString=a  ID=bus277  Vbase=110000  Vref=1  Vangle=0  VLF=1  angleLF=0
      settings: AttributesFormatString=|
      | %<ID>
      | %<Vbase>V
      | %<VLF>pu
      | %<angleLF>deg.
      | %<Name>
  bus278 : powerlib/Measurements/Load Flow Bus  LConnTagsString=a  ID=bus278  Vbase=110000  Vref=1  Vangle=0  VLF=1  angleLF=0
      settings: AttributesFormatString=|
      | %<ID>
      | %<Vbase>V
      | %<VLF>pu
      | %<angleLF>deg.
      | %<Name>
  bus279 : powerlib/Measurements/Load Flow Bus  LConnTagsString=a  ID=bus279  Vbase=110000  Vref=1  Vangle=0  VLF=1  angleLF=0
      settings: AttributesFormatString=|
      | %<ID>
      | %<Vbase>V
      | %<VLF>pu
      | %<angleLF>deg.
      | %<Name>
  bus28 : powerlib/Measurements/Load Flow Bus  LConnTagsString=a  ID=bus28  Vbase=110000  Vref=1  Vangle=0  VLF=1  angleLF=0
      settings: AttributesFormatString=|
      | %<ID>
      | %<Vbase>V
      | %<VLF>pu
      | %<angleLF>deg.
      | %<Name>
  bus280 : powerlib/Measurements/Load Flow Bus  LConnTagsString=a  ID=bus280  Vbase=110000  Vref=1  Vangle=0  VLF=1  angleLF=0
      settings: AttributesFormatString=|
      | %<ID>
      | %<Vbase>V
      | %<VLF>pu
      | %<angleLF>deg.
      | %<Name>
  bus281 : powerlib/Measurements/Load Flow Bus  LConnTagsString=a  ID=bus281  Vbase=110000  Vref=1  Vangle=0  VLF=1  angleLF=0
      settings: AttributesFormatString=|
      | %<ID>
      | %<Vbase>V
      | %<VLF>pu
      | %<angleLF>deg.
      | %<Name>
  bus282 : powerlib/Measurements/Load Flow Bus  LConnTagsString=a  ID=bus282  Vbase=110000  Vref=1  Vangle=0  VLF=1  angleLF=0
      settings: AttributesFormatString=|
      | %<ID>
      | %<Vbase>V
      | %<VLF>pu
      | %<angleLF>deg.
      | %<Name>
  bus283 : powerlib/Measurements/Load Flow Bus  LConnTagsString=a  ID=bus283  Vbase=110000  Vref=1  Vangle=0  VLF=1  angleLF=0
      settings: AttributesFormatString=|
      | %<ID>
      | %<Vbase>V
      | %<VLF>pu
      | %<angleLF>deg.
      | %<Name>
  bus284 : powerlib/Measurements/Load Flow Bus  LConnTagsString=a  ID=bus284  Vbase=110000  Vref=1  Vangle=0  VLF=1  angleLF=0
      settings: AttributesFormatString=|
      | %<ID>
      | %<Vbase>V
      | %<VLF>pu
      | %<angleLF>deg.
      | %<Name>
  bus285 : powerlib/Measurements/Load Flow Bus  LConnTagsString=a  ID=bus285  Vbase=110000  Vref=1  Vangle=0  VLF=1  angleLF=0
      settings: AttributesFormatString=|
      | %<ID>
      | %<Vbase>V
      | %<VLF>pu
      | %<angleLF>deg.
      | %<Name>
  bus286 : powerlib/Measurements/Load Flow Bus  LConnTagsString=a  ID=bus286  Vbase=110000  Vref=1  Vangle=0  VLF=1  angleLF=0
      settings: AttributesFormatString=|
      | %<ID>
      | %<Vbase>V
      | %<VLF>pu
      | %<angleLF>deg.
      | %<Name>
  bus287 : powerlib/Measurements/Load Flow Bus  LConnTagsString=a  ID=bus287  Vbase=110000  Vref=1  Vangle=0  VLF=1  angleLF=0
      settings: AttributesFormatString=|
      | %<ID>
      | %<Vbase>V
      | %<VLF>pu
      | %<angleLF>deg.
      | %<Name>
  bus288 : powerlib/Measurements/Load Flow Bus  LConnTagsString=a  ID=bus288  Vbase=110000  Vref=1  Vangle=0  VLF=1  angleLF=0
      settings: AttributesFormatString=|
      | %<ID>
      | %<Vbase>V
      | %<VLF>pu
      | %<angleLF>deg.
      | %<Name>
  bus289 : powerlib/Measurements/Load Flow Bus  LConnTagsString=a  ID=bus289  Vbase=110000  Vref=1  Vangle=0  VLF=1  angleLF=0
      settings: AttributesFormatString=|
      | %<ID>
      | %<Vbase>V
      | %<VLF>pu
      | %<angleLF>deg.
      | %<Name>
  bus29 : powerlib/Measurements/Load Flow Bus  LConnTagsString=a  ID=bus29  Vbase=110000  Vref=1  Vangle=0  VLF=1  angleLF=0
      settings: AttributesFormatString=|
      | %<ID>
      | %<Vbase>V
      | %<VLF>pu
      | %<angleLF>deg.
      | %<Name>
  bus290 : powerlib/Measurements/Load Flow Bus  LConnTagsString=a  ID=bus290  Vbase=110000  Vref=1  Vangle=0  VLF=1  angleLF=0
      settings: AttributesFormatString=|
      | %<ID>
      | %<Vbase>V
      | %<VLF>pu
      | %<angleLF>deg.
      | %<Name>
  bus291 : powerlib/Measurements/Load Flow Bus  LConnTagsString=a  ID=bus291  Vbase=110000  Vref=1  Vangle=0  VLF=1  angleLF=0
      settings: AttributesFormatString=|
      | %<ID>
      | %<Vbase>V
      | %<VLF>pu
      | %<angleLF>deg.
      | %<Name>
  bus292 : powerlib/Measurements/Load Flow Bus  LConnTagsString=a  ID=bus292  Vbase=110000  Vref=1  Vangle=0  VLF=1  angleLF=0
      settings: AttributesFormatString=|
      | %<ID>
      | %<Vbase>V
      | %<VLF>pu
      | %<angleLF>deg.
      | %<Name>
  bus293 : powerlib/Measurements/Load Flow Bus  LConnTagsString=a  ID=bus293  Vbase=110000  Vref=1  Vangle=0  VLF=1  angleLF=0
      settings: AttributesFormatString=|
      | %<ID>
      | %<Vbase>V
      | %<VLF>pu
      | %<angleLF>deg.
      | %<Name>
  bus294 : powerlib/Measurements/Load Flow Bus  LConnTagsString=a  ID=bus294  Vbase=110000  Vref=1  Vangle=0  VLF=1  angleLF=0
      settings: AttributesFormatString=|
      | %<ID>
      | %<Vbase>V
      | %<VLF>pu
      | %<angleLF>deg.
      | %<Name>
  bus295 : powerlib/Measurements/Load Flow Bus  LConnTagsString=a  ID=bus295  Vbase=110000  Vref=1  Vangle=0  VLF=1  angleLF=0
      settings: AttributesFormatString=|
      | %<ID>
      | %<Vbase>V
      | %<VLF>pu
      | %<angleLF>deg.
      | %<Name>
  bus296 : powerlib/Measurements/Load Flow Bus  LConnTagsString=a  ID=bus296  Vbase=110000  Vref=1  Vangle=0  VLF=1  angleLF=0
      settings: AttributesFormatString=|
      | %<ID>
      | %<Vbase>V
      | %<VLF>pu
      | %<angleLF>deg.
      | %<Name>
  bus297 : powerlib/Measurements/Load Flow Bus  LConnTagsString=a  ID=bus297  Vbase=110000  Vref=1  Vangle=0  VLF=1  angleLF=0
      settings: AttributesFormatString=|
      | %<ID>
      | %<Vbase>V
      | %<VLF>pu
      | %<angleLF>deg.
      | %<Name>
  bus298 : powerlib/Measurements/Load Flow Bus  LConnTagsString=a  ID=bus298  Vbase=110000  Vref=1  Vangle=0  VLF=1  angleLF=0
      settings: AttributesFormatString=|
      | %<ID>
      | %<Vbase>V
      | %<VLF>pu
      | %<angleLF>deg.
      | %<Name>
  bus299 : powerlib/Measurements/Load Flow Bus  LConnTagsString=a  ID=bus299  Vbase=110000  Vref=1  Vangle=0  VLF=1  angleLF=0
      settings: AttributesFormatString=|
      | %<ID>
      | %<Vbase>V
      | %<VLF>pu
      | %<angleLF>deg.
      | %<Name>
  bus3 : powerlib/Measurements/Load Flow Bus  LConnTagsString=a  ID=bus3  Vbase=110000  Vref=1  Vangle=0  VLF=1  angleLF=0
      settings: AttributesFormatString=|
      | %<ID>
      | %<Vbase>V
      | %<VLF>pu
      | %<angleLF>deg.
      | %<Name>
  bus30 : powerlib/Measurements/Load Flow Bus  LConnTagsString=a  ID=bus30  Vbase=110000  Vref=1  Vangle=0  VLF=1  angleLF=0
      settings: AttributesFormatString=|
      | %<ID>
      | %<Vbase>V
      | %<VLF>pu
      | %<angleLF>deg.
      | %<Name>
  bus300 : powerlib/Measurements/Load Flow Bus  LConnTagsString=a  ID=bus300  Vbase=110000  Vref=1  Vangle=0  VLF=1  angleLF=0
      settings: AttributesFormatString=|
      | %<ID>
      | %<Vbase>V
      | %<VLF>pu
      | %<angleLF>deg.
      | %<Name>
  bus301 : powerlib/Measurements/Load Flow Bus  LConnTagsString=a  ID=bus301  Vbase=110000  Vref=1  Vangle=0  VLF=1  angleLF=0
      settings: AttributesFormatString=|
      | %<ID>
      | %<Vbase>V
      | %<VLF>pu
      | %<angleLF>deg.
      | %<Name>
  bus302 : powerlib/Measurements/Load Flow Bus  LConnTagsString=a  ID=bus302  Vbase=110000  Vref=1  Vangle=0  VLF=1  angleLF=0
      settings: AttributesFormatString=|
      | %<ID>
      | %<Vbase>V
      | %<VLF>pu
      | %<angleLF>deg.
      | %<Name>
  bus303 : powerlib/Measurements/Load Flow Bus  LConnTagsString=a  ID=bus303  Vbase=110000  Vref=1  Vangle=0  VLF=1  angleLF=0
      settings: AttributesFormatString=|
      | %<ID>
      | %<Vbase>V
      | %<VLF>pu
      | %<angleLF>deg.
      | %<Name>
  bus304 : powerlib/Measurements/Load Flow Bus  LConnTagsString=a  ID=bus304  Vbase=110000  Vref=1  Vangle=0  VLF=1  angleLF=0
      settings: AttributesFormatString=|
      | %<ID>
      | %<Vbase>V
      | %<VLF>pu
      | %<angleLF>deg.
      | %<Name>
  bus305 : powerlib/Measurements/Load Flow Bus  LConnTagsString=a  ID=bus305  Vbase=110000  Vref=1  Vangle=0  VLF=1  angleLF=0
      settings: AttributesFormatString=|
      | %<ID>
      | %<Vbase>V
      | %<VLF>pu
      | %<angleLF>deg.
      | %<Name>
  bus306 : powerlib/Measurements/Load Flow Bus  LConnTagsString=a  ID=bus306  Vbase=110000  Vref=1  Vangle=0  VLF=1  angleLF=0
      settings: AttributesFormatString=|
      | %<ID>
      | %<Vbase>V
      | %<VLF>pu
      | %<angleLF>deg.
      | %<Name>
  bus307 : powerlib/Measurements/Load Flow Bus  LConnTagsString=a  ID=bus307  Vbase=110000  Vref=1  Vangle=0  VLF=1  angleLF=0
      settings: AttributesFormatString=|
      | %<ID>
      | %<Vbase>V
      | %<VLF>pu
      | %<angleLF>deg.
      | %<Name>
  bus308 : powerlib/Measurements/Load Flow Bus  LConnTagsString=a  ID=bus308  Vbase=110000  Vref=1  Vangle=0  VLF=1  angleLF=0
      settings: AttributesFormatString=|
      | %<ID>
      | %<Vbase>V
      | %<VLF>pu
      | %<angleLF>deg.
      | %<Name>
  bus309 : powerlib/Measurements/Load Flow Bus  LConnTagsString=a  ID=bus309  Vbase=110000  Vref=1  Vangle=0  VLF=1  angleLF=0
      settings: AttributesFormatString=|
      | %<ID>
      | %<Vbase>V
      | %<VLF>pu
      | %<angleLF>deg.
      | %<Name>
  bus31 : powerlib/Measurements/Load Flow Bus  LConnTagsString=a  ID=bus31  Vbase=110000  Vref=1  Vangle=0  VLF=1  angleLF=0
      settings: AttributesFormatString=|
      | %<ID>
      | %<Vbase>V
      | %<VLF>pu
      | %<angleLF>deg.
      | %<Name>
  bus310 : powerlib/Measurements/Load Flow Bus  LConnTagsString=a  ID=bus310  Vbase=110000  Vref=1  Vangle=0  VLF=1  angleLF=0
      settings: AttributesFormatString=|
      | %<ID>
      | %<Vbase>V
      | %<VLF>pu
      | %<angleLF>deg.
      | %<Name>
  bus311 : powerlib/Measurements/Load Flow Bus  LConnTagsString=a  ID=bus311  Vbase=110000  Vref=1  Vangle=0  VLF=1  angleLF=0
      settings: AttributesFormatString=|
      | %<ID>
      | %<Vbase>V
      | %<VLF>pu
      | %<angleLF>deg.
      | %<Name>
  bus312 : powerlib/Measurements/Load Flow Bus  LConnTagsString=a  ID=bus312  Vbase=110000  Vref=1  Vangle=0  VLF=1  angleLF=0
      settings: AttributesFormatString=|
      | %<ID>
      | %<Vbase>V
      | %<VLF>pu
      | %<angleLF>deg.
      | %<Name>
  bus313 : powerlib/Measurements/Load Flow Bus  LConnTagsString=a  ID=bus313  Vbase=110000  Vref=1  Vangle=0  VLF=1  angleLF=0
      settings: AttributesFormatString=|
      | %<ID>
      | %<Vbase>V
      | %<VLF>pu
      | %<angleLF>deg.
      | %<Name>
  bus314 : powerlib/Measurements/Load Flow Bus  LConnTagsString=a  ID=bus314  Vbase=110000  Vref=1  Vangle=0  VLF=1  angleLF=0
      settings: AttributesFormatString=|
      | %<ID>
      | %<Vbase>V
      | %<VLF>pu
      | %<angleLF>deg.
      | %<Name>
  bus315 : powerlib/Measurements/Load Flow Bus  LConnTagsString=a  ID=bus315  Vbase=110000  Vref=1  Vangle=0  VLF=1  angleLF=0
      settings: AttributesFormatString=|
      | %<ID>
      | %<Vbase>V
      | %<VLF>pu
      | %<angleLF>deg.
      | %<Name>
  bus316 : powerlib/Measurements/Load Flow Bus  LConnTagsString=a  ID=bus316  Vbase=110000  Vref=1  Vangle=0  VLF=1  angleLF=0
      settings: AttributesFormatString=|
      | %<ID>
      | %<Vbase>V
      | %<VLF>pu
      | %<angleLF>deg.
      | %<Name>
  bus317 : powerlib/Measurements/Load Flow Bus  LConnTagsString=a  ID=bus317  Vbase=110000  Vref=1  Vangle=0  VLF=1  angleLF=0
      settings: AttributesFormatString=|
      | %<ID>
      | %<Vbase>V
      | %<VLF>pu
      | %<angleLF>deg.
      | %<Name>
  bus318 : powerlib/Measurements/Load Flow Bus  LConnTagsString=a  ID=bus318  Vbase=110000  Vref=1  Vangle=0  VLF=1  angleLF=0
      settings: AttributesFormatString=|
      | %<ID>
      | %<Vbase>V
      | %<VLF>pu
      | %<angleLF>deg.
      | %<Name>
  bus319 : powerlib/Measurements/Load Flow Bus  LConnTagsString=a  ID=bus319  Vbase=110000  Vref=1  Vangle=0  VLF=1  angleLF=0
      settings: AttributesFormatString=|
      | %<ID>
      | %<Vbase>V
      | %<VLF>pu
      | %<angleLF>deg.
      | %<Name>
  bus32 : powerlib/Measurements/Load Flow Bus  LConnTagsString=a  ID=bus32  Vbase=110000  Vref=1  Vangle=0  VLF=1  angleLF=0
      settings: AttributesFormatString=|
      | %<ID>
      | %<Vbase>V
      | %<VLF>pu
      | %<angleLF>deg.
      | %<Name>
  bus320 : powerlib/Measurements/Load Flow Bus  LConnTagsString=a  ID=bus320  Vbase=110000  Vref=1  Vangle=0  VLF=1  angleLF=0
      settings: AttributesFormatString=|
      | %<ID>
      | %<Vbase>V
      | %<VLF>pu
      | %<angleLF>deg.
      | %<Name>
  bus321 : powerlib/Measurements/Load Flow Bus  LConnTagsString=a  ID=bus321  Vbase=110000  Vref=1  Vangle=0  VLF=1  angleLF=0
      settings: AttributesFormatString=|
      | %<ID>
      | %<Vbase>V
      | %<VLF>pu
      | %<angleLF>deg.
      | %<Name>
  bus322 : powerlib/Measurements/Load Flow Bus  LConnTagsString=a  ID=bus322  Vbase=110000  Vref=1  Vangle=0  VLF=1  angleLF=0
      settings: AttributesFormatString=|
      | %<ID>
      | %<Vbase>V
      | %<VLF>pu
      | %<angleLF>deg.
      | %<Name>
  bus323 : powerlib/Measurements/Load Flow Bus  LConnTagsString=a  ID=bus323  Vbase=110000  Vref=1  Vangle=0  VLF=1  angleLF=0
      settings: AttributesFormatString=|
      | %<ID>
      | %<Vbase>V
      | %<VLF>pu
      | %<angleLF>deg.
      | %<Name>
  bus324 : powerlib/Measurements/Load Flow Bus  LConnTagsString=a  ID=bus324  Vbase=110000  Vref=1  Vangle=0  VLF=1  angleLF=0
      settings: AttributesFormatString=|
      | %<ID>
      | %<Vbase>V
      | %<VLF>pu
      | %<angleLF>deg.
      | %<Name>
  bus325 : powerlib/Measurements/Load Flow Bus  LConnTagsString=a  ID=bus325  Vbase=110000  Vref=1  Vangle=0  VLF=1  angleLF=0
      settings: AttributesFormatString=|
      | %<ID>
      | %<Vbase>V
      | %<VLF>pu
      | %<angleLF>deg.
      | %<Name>
  bus326 : powerlib/Measurements/Load Flow Bus  LConnTagsString=a  ID=bus326  Vbase=110000  Vref=1  Vangle=0  VLF=1  angleLF=0
      settings: AttributesFormatString=|
      | %<ID>
      | %<Vbase>V
      | %<VLF>pu
      | %<angleLF>deg.
      | %<Name>
  bus327 : powerlib/Measurements/Load Flow Bus  LConnTagsString=a  ID=bus327  Vbase=110000  Vref=1  Vangle=0  VLF=1  angleLF=0
      settings: AttributesFormatString=|
      | %<ID>
      | %<Vbase>V
      | %<VLF>pu
      | %<angleLF>deg.
      | %<Name>
  bus328 : powerlib/Measurements/Load Flow Bus  LConnTagsString=a  ID=bus328  Vbase=110000  Vref=1  Vangle=0  VLF=1  angleLF=0
      settings: AttributesFormatString=|
      | %<ID>
      | %<Vbase>V
      | %<VLF>pu
      | %<angleLF>deg.
      | %<Name>
  bus329 : powerlib/Measurements/Load Flow Bus  LConnTagsString=a  ID=bus329  Vbase=110000  Vref=1  Vangle=0  VLF=1  angleLF=0
      settings: AttributesFormatString=|
      | %<ID>
      | %<Vbase>V
      | %<VLF>pu
      | %<angleLF>deg.
      | %<Name>
  bus33 : powerlib/Measurements/Load Flow Bus  LConnTagsString=a  ID=bus33  Vbase=110000  Vref=1  Vangle=0  VLF=1  angleLF=0
      settings: AttributesFormatString=|
      | %<ID>
      | %<Vbase>V
      | %<VLF>pu
      | %<angleLF>deg.
      | %<Name>
  bus330 : powerlib/Measurements/Load Flow Bus  LConnTagsString=a  ID=bus330  Vbase=110000  Vref=1  Vangle=0  VLF=1  angleLF=0
      settings: AttributesFormatString=|
      | %<ID>
      | %<Vbase>V
      | %<VLF>pu
      | %<angleLF>deg.
      | %<Name>
  bus331 : powerlib/Measurements/Load Flow Bus  LConnTagsString=a  ID=bus331  Vbase=110000  Vref=1  Vangle=0  VLF=1  angleLF=0
      settings: AttributesFormatString=|
      | %<ID>
      | %<Vbase>V
      | %<VLF>pu
      | %<angleLF>deg.
      | %<Name>
  bus332 : powerlib/Measurements/Load Flow Bus  LConnTagsString=a  ID=bus332  Vbase=110000  Vref=1  Vangle=0  VLF=1  angleLF=0
      settings: AttributesFormatString=|
      | %<ID>
      | %<Vbase>V
      | %<VLF>pu
      | %<angleLF>deg.
      | %<Name>
  bus333 : powerlib/Measurements/Load Flow Bus  LConnTagsString=a  ID=bus333  Vbase=110000  Vref=1  Vangle=0  VLF=1  angleLF=0
      settings: AttributesFormatString=|
      | %<ID>
      | %<Vbase>V
      | %<VLF>pu
      | %<angleLF>deg.
      | %<Name>
  bus334 : powerlib/Measurements/Load Flow Bus  LConnTagsString=a  ID=bus334  Vbase=110000  Vref=1  Vangle=0  VLF=1  angleLF=0
      settings: AttributesFormatString=|
      | %<ID>
      | %<Vbase>V
      | %<VLF>pu
      | %<angleLF>deg.
      | %<Name>
  bus335 : powerlib/Measurements/Load Flow Bus  LConnTagsString=a  ID=bus335  Vbase=110000  Vref=1  Vangle=0  VLF=1  angleLF=0
      settings: AttributesFormatString=|
      | %<ID>
      | %<Vbase>V
      | %<VLF>pu
      | %<angleLF>deg.
      | %<Name>
  bus336 : powerlib/Measurements/Load Flow Bus  LConnTagsString=a  ID=bus336  Vbase=110000  Vref=1  Vangle=0  VLF=1  angleLF=0
      settings: AttributesFormatString=|
      | %<ID>
      | %<Vbase>V
      | %<VLF>pu
      | %<angleLF>deg.
      | %<Name>
  bus337 : powerlib/Measurements/Load Flow Bus  LConnTagsString=a  ID=bus337  Vbase=110000  Vref=1  Vangle=0  VLF=1  angleLF=0
      settings: AttributesFormatString=|
      | %<ID>
      | %<Vbase>V
      | %<VLF>pu
      | %<angleLF>deg.
      | %<Name>
  bus338 : powerlib/Measurements/Load Flow Bus  LConnTagsString=a  ID=bus338  Vbase=110000  Vref=1  Vangle=0  VLF=1  angleLF=0
      settings: AttributesFormatString=|
      | %<ID>
      | %<Vbase>V
      | %<VLF>pu
      | %<angleLF>deg.
      | %<Name>
  bus339 : powerlib/Measurements/Load Flow Bus  LConnTagsString=a  ID=bus339  Vbase=110000  Vref=1  Vangle=0  VLF=1  angleLF=0
      settings: AttributesFormatString=|
      | %<ID>
      | %<Vbase>V
      | %<VLF>pu
      | %<angleLF>deg.
      | %<Name>
  bus34 : powerlib/Measurements/Load Flow Bus  LConnTagsString=a  ID=bus34  Vbase=110000  Vref=1  Vangle=0  VLF=1  angleLF=0
      settings: AttributesFormatString=|
      | %<ID>
      | %<Vbase>V
      | %<VLF>pu
      | %<angleLF>deg.
      | %<Name>
  bus340 : powerlib/Measurements/Load Flow Bus  LConnTagsString=a  ID=bus340  Vbase=110000  Vref=1  Vangle=0  VLF=1  angleLF=0
      settings: AttributesFormatString=|
      | %<ID>
      | %<Vbase>V
      | %<VLF>pu
      | %<angleLF>deg.
      | %<Name>
  bus341 : powerlib/Measurements/Load Flow Bus  LConnTagsString=a  ID=bus341  Vbase=110000  Vref=1  Vangle=0  VLF=1  angleLF=0
      settings: AttributesFormatString=|
      | %<ID>
      | %<Vbase>V
      | %<VLF>pu
      | %<angleLF>deg.
      | %<Name>
  bus342 : powerlib/Measurements/Load Flow Bus  LConnTagsString=a  ID=bus342  Vbase=110000  Vref=1  Vangle=0  VLF=1  angleLF=0
      settings: AttributesFormatString=|
      | %<ID>
      | %<Vbase>V
      | %<VLF>pu
      | %<angleLF>deg.
      | %<Name>
  bus343 : powerlib/Measurements/Load Flow Bus  LConnTagsString=a  ID=bus343  Vbase=220000  Vref=1  Vangle=0  VLF=1  angleLF=0
      settings: AttributesFormatString=|
      | %<ID>
      | %<Vbase>V
      | %<VLF>pu
      | %<angleLF>deg.
      | %<Name>
  bus344 : powerlib/Measurements/Load Flow Bus  LConnTagsString=a  ID=bus344  Vbase=220000  Vref=1  Vangle=0  VLF=1  angleLF=0
      settings: AttributesFormatString=|
      | %<ID>
      | %<Vbase>V
      | %<VLF>pu
      | %<angleLF>deg.
      | %<Name>
  bus345 : powerlib/Measurements/Load Flow Bus  LConnTagsString=a  ID=bus345  Vbase=220000  Vref=1  Vangle=0  VLF=1  angleLF=0
      settings: AttributesFormatString=|
      | %<ID>
      | %<Vbase>V
      | %<VLF>pu
      | %<angleLF>deg.
      | %<Name>
  bus346 : powerlib/Measurements/Load Flow Bus  LConnTagsString=a  ID=bus346  Vbase=220000  Vref=1  Vangle=0  VLF=1  angleLF=0
      settings: AttributesFormatString=|
      | %<ID>
      | %<Vbase>V
      | %<VLF>pu
      | %<angleLF>deg.
      | %<Name>
  bus347 : powerlib/Measurements/Load Flow Bus  LConnTagsString=a  ID=bus347  Vbase=220000  Vref=1  Vangle=0  VLF=1  angleLF=0
      settings: AttributesFormatString=|
      | %<ID>
      | %<Vbase>V
      | %<VLF>pu
      | %<angleLF>deg.
      | %<Name>
  bus348 : powerlib/Measurements/Load Flow Bus  LConnTagsString=a  ID=bus348  Vbase=220000  Vref=1  Vangle=0  VLF=1  angleLF=0
      settings: AttributesFormatString=|
      | %<ID>
      | %<Vbase>V
      | %<VLF>pu
      | %<angleLF>deg.
      | %<Name>
  bus349 : powerlib/Measurements/Load Flow Bus  LConnTagsString=a  ID=bus349  Vbase=220000  Vref=1  Vangle=0  VLF=1  angleLF=0
      settings: AttributesFormatString=|
      | %<ID>
      | %<Vbase>V
      | %<VLF>pu
      | %<angleLF>deg.
      | %<Name>
  bus35 : powerlib/Measurements/Load Flow Bus  LConnTagsString=a  ID=bus35  Vbase=110000  Vref=1  Vangle=0  VLF=1  angleLF=0
      settings: AttributesFormatString=|
      | %<ID>
      | %<Vbase>V
      | %<VLF>pu
      | %<angleLF>deg.
      | %<Name>
  bus350 : powerlib/Measurements/Load Flow Bus  LConnTagsString=a  ID=bus350  Vbase=220000  Vref=1  Vangle=0  VLF=1  angleLF=0
      settings: AttributesFormatString=|
      | %<ID>
      | %<Vbase>V
      | %<VLF>pu
      | %<angleLF>deg.
      | %<Name>
  bus351 : powerlib/Measurements/Load Flow Bus  LConnTagsString=a  ID=bus351  Vbase=220000  Vref=1  Vangle=0  VLF=1  angleLF=0
      settings: AttributesFormatString=|
      | %<ID>
      | %<Vbase>V
      | %<VLF>pu
      | %<angleLF>deg.
      | %<Name>
  bus352 : powerlib/Measurements/Load Flow Bus  LConnTagsString=a  ID=bus352  Vbase=220000  Vref=1  Vangle=0  VLF=1  angleLF=0
      settings: AttributesFormatString=|
      | %<ID>
      | %<Vbase>V
      | %<VLF>pu
      | %<angleLF>deg.
      | %<Name>
  bus353 : powerlib/Measurements/Load Flow Bus  LConnTagsString=a  ID=bus353  Vbase=220000  Vref=1  Vangle=0  VLF=1  angleLF=0
      settings: AttributesFormatString=|
      | %<ID>
      | %<Vbase>V
      | %<VLF>pu
      | %<angleLF>deg.
      | %<Name>
  bus354 : powerlib/Measurements/Load Flow Bus  LConnTagsString=a  ID=bus354  Vbase=220000  Vref=1  Vangle=0  VLF=1  angleLF=0
      settings: AttributesFormatString=|
      | %<ID>
      | %<Vbase>V
      | %<VLF>pu
      | %<angleLF>deg.
      | %<Name>
  bus355 : powerlib/Measurements/Load Flow Bus  LConnTagsString=a  ID=bus355  Vbase=220000  Vref=1  Vangle=0  VLF=1  angleLF=0
      settings: AttributesFormatString=|
      | %<ID>
      | %<Vbase>V
      | %<VLF>pu
      | %<angleLF>deg.
      | %<Name>
  bus356 : powerlib/Measurements/Load Flow Bus  LConnTagsString=a  ID=bus356  Vbase=220000  Vref=1  Vangle=0  VLF=1  angleLF=0
      settings: AttributesFormatString=|
      | %<ID>
      | %<Vbase>V
      | %<VLF>pu
      | %<angleLF>deg.
      | %<Name>
  bus357 : powerlib/Measurements/Load Flow Bus  LConnTagsString=a  ID=bus357  Vbase=220000  Vref=1  Vangle=0  VLF=1  angleLF=0
      settings: AttributesFormatString=|
      | %<ID>
      | %<Vbase>V
      | %<VLF>pu
      | %<angleLF>deg.
      | %<Name>
  bus358 : powerlib/Measurements/Load Flow Bus  LConnTagsString=a  ID=bus358  Vbase=220000  Vref=1  Vangle=0  VLF=1  angleLF=0
      settings: AttributesFormatString=|
      | %<ID>
      | %<Vbase>V
      | %<VLF>pu
      | %<angleLF>deg.
      | %<Name>
  bus359 : powerlib/Measurements/Load Flow Bus  LConnTagsString=a  ID=bus359  Vbase=220000  Vref=1  Vangle=0  VLF=1  angleLF=0
      settings: AttributesFormatString=|
      | %<ID>
      | %<Vbase>V
      | %<VLF>pu
      | %<angleLF>deg.
      | %<Name>
  bus36 : powerlib/Measurements/Load Flow Bus  LConnTagsString=a  ID=bus36  Vbase=110000  Vref=1  Vangle=0  VLF=1  angleLF=0
      settings: AttributesFormatString=|
      | %<ID>
      | %<Vbase>V
      | %<VLF>pu
      | %<angleLF>deg.
      | %<Name>
  bus360 : powerlib/Measurements/Load Flow Bus  LConnTagsString=a  ID=bus360  Vbase=220000  Vref=1  Vangle=0  VLF=1  angleLF=0
      settings: AttributesFormatString=|
      | %<ID>
      | %<Vbase>V
      | %<VLF>pu
      | %<angleLF>deg.
      | %<Name>
  bus361 : powerlib/Measurements/Load Flow Bus  LConnTagsString=a  ID=bus361  Vbase=220000  Vref=1  Vangle=0  VLF=1  angleLF=0
      settings: AttributesFormatString=|
      | %<ID>
      | %<Vbase>V
      | %<VLF>pu
      | %<angleLF>deg.
      | %<Name>
  bus362 : powerlib/Measurements/Load Flow Bus  LConnTagsString=a  ID=bus362  Vbase=220000  Vref=1  Vangle=0  VLF=1  angleLF=0
      settings: AttributesFormatString=|
      | %<ID>
      | %<Vbase>V
      | %<VLF>pu
      | %<angleLF>deg.
      | %<Name>
  bus363 : powerlib/Measurements/Load Flow Bus  LConnTagsString=a  ID=bus363  Vbase=220000  Vref=1  Vangle=0  VLF=1  angleLF=0
      settings: AttributesFormatString=|
      | %<ID>
      | %<Vbase>V
      | %<VLF>pu
      | %<angleLF>deg.
      | %<Name>
  bus364 : powerlib/Measurements/Load Flow Bus  LConnTagsString=a  ID=bus364  Vbase=500000  Vref=1  Vangle=0  VLF=1  angleLF=0
      settings: AttributesFormatString=|
      | %<ID>
      | %<Vbase>V
      | %<VLF>pu
      | %<angleLF>deg.
      | %<Name>
  bus365 : powerlib/Measurements/Load Flow Bus  LConnTagsString=a  ID=bus365  Vbase=500000  Vref=1  Vangle=0  VLF=1  angleLF=0
      settings: AttributesFormatString=|
      | %<ID>
      | %<Vbase>V
      | %<VLF>pu
      | %<angleLF>deg.
      | %<Name>
  bus366 : powerlib/Measurements/Load Flow Bus  LConnTagsString=a  ID=bus366  Vbase=500000  Vref=1  Vangle=0  VLF=1  angleLF=0
      settings: AttributesFormatString=|
      | %<ID>
      | %<Vbase>V
      | %<VLF>pu
      | %<angleLF>deg.
      | %<Name>
  bus367 : powerlib/Measurements/Load Flow Bus  LConnTagsString=a  ID=bus367  Vbase=500000  Vref=1  Vangle=0  VLF=1  angleLF=0
      settings: AttributesFormatString=|
      | %<ID>
      | %<Vbase>V
      | %<VLF>pu
      | %<angleLF>deg.
      | %<Name>
  bus368 : powerlib/Measurements/Load Flow Bus  LConnTagsString=a  ID=bus368  Vbase=500000  Vref=1  Vangle=0  VLF=1  angleLF=0
      settings: AttributesFormatString=|
      | %<ID>
      | %<Vbase>V
      | %<VLF>pu
      | %<angleLF>deg.
      | %<Name>
  bus369 : powerlib/Measurements/Load Flow Bus  LConnTagsString=a  ID=bus369  Vbase=500000  Vref=1  Vangle=0  VLF=1  angleLF=0
      settings: AttributesFormatString=|
      | %<ID>
      | %<Vbase>V
      | %<VLF>pu
      | %<angleLF>deg.
      | %<Name>
  bus37 : powerlib/Measurements/Load Flow Bus  LConnTagsString=a  ID=bus37  Vbase=110000  Vref=1  Vangle=0  VLF=1  angleLF=0
      settings: AttributesFormatString=|
      | %<ID>
      | %<Vbase>V
      | %<VLF>pu
      | %<angleLF>deg.
      | %<Name>
  bus370 : powerlib/Measurements/Load Flow Bus  LConnTagsString=a  ID=bus370  Vbase=500000  Vref=1  Vangle=0  VLF=1  angleLF=0
      settings: AttributesFormatString=|
      | %<ID>
      | %<Vbase>V
      | %<VLF>pu
      | %<angleLF>deg.
      | %<Name>
  bus371 : powerlib/Measurements/Load Flow Bus  LConnTagsString=a  ID=bus371  Vbase=500000  Vref=1  Vangle=0  VLF=1  angleLF=0
      settings: AttributesFormatString=|
      | %<ID>
      | %<Vbase>V
      | %<VLF>pu
      | %<angleLF>deg.
      | %<Name>
  bus372 : powerlib/Measurements/Load Flow Bus  LConnTagsString=a  ID=bus372  Vbase=500000  Vref=1  Vangle=0  VLF=1  angleLF=0
      settings: AttributesFormatString=|
      | %<ID>
      | %<Vbase>V
      | %<VLF>pu
      | %<angleLF>deg.
      | %<Name>
  bus373 : powerlib/Measurements/Load Flow Bus  LConnTagsString=a  ID=bus373  Vbase=500000  Vref=1  Vangle=0  VLF=1  angleLF=0
      settings: AttributesFormatString=|
      | %<ID>
      | %<Vbase>V
      | %<VLF>pu
      | %<angleLF>deg.
      | %<Name>
  bus374 : powerlib/Measurements/Load Flow Bus  LConnTagsString=a  ID=bus374  Vbase=500000  Vref=1  Vangle=0  VLF=1  angleLF=0
      settings: AttributesFormatString=|
      | %<ID>
      | %<Vbase>V
      | %<VLF>pu
      | %<angleLF>deg.
      | %<Name>
  bus375 : powerlib/Measurements/Load Flow Bus  LConnTagsString=a  ID=bus375  Vbase=500000  Vref=1  Vangle=0  VLF=1  angleLF=0
      settings: AttributesFormatString=|
      | %<ID>
      | %<Vbase>V
      | %<VLF>pu
      | %<angleLF>deg.
      | %<Name>
  bus376 : powerlib/Measurements/Load Flow Bus  LConnTagsString=a  ID=bus376  Vbase=500000  Vref=1  Vangle=0  VLF=1  angleLF=0
      settings: AttributesFormatString=|
      | %<ID>
      | %<Vbase>V
      | %<VLF>pu
      | %<angleLF>deg.
      | %<Name>
  bus377 : powerlib/Measurements/Load Flow Bus  LConnTagsString=a  ID=bus377  Vbase=500000  Vref=1  Vangle=0  VLF=1  angleLF=0
      settings: AttributesFormatString=|
      | %<ID>
      | %<Vbase>V
      | %<VLF>pu
      | %<angleLF>deg.
      | %<Name>
  bus378 : powerlib/Measurements/Load Flow Bus  LConnTagsString=a  ID=bus378  Vbase=500000  Vref=1  Vangle=0  VLF=1  angleLF=0
      settings: AttributesFormatString=|
      | %<ID>
      | %<Vbase>V
      | %<VLF>pu
      | %<angleLF>deg.
      | %<Name>
  bus38 : powerlib/Measurements/Load Flow Bus  LConnTagsString=a  ID=bus38  Vbase=110000  Vref=1  Vangle=0  VLF=1  angleLF=0
      settings: AttributesFormatString=|
      | %<ID>
      | %<Vbase>V
      | %<VLF>pu
      | %<angleLF>deg.
      | %<Name>
  bus39 : powerlib/Measurements/Load Flow Bus  LConnTagsString=a  ID=bus39  Vbase=110000  Vref=1  Vangle=0  VLF=1  angleLF=0
      settings: AttributesFormatString=|
      | %<ID>
      | %<Vbase>V
      | %<VLF>pu
      | %<angleLF>deg.
      | %<Name>
  bus4 : powerlib/Measurements/Load Flow Bus  LConnTagsString=a  ID=bus4  Vbase=110000  Vref=1  Vangle=0  VLF=1  angleLF=0
      settings: AttributesFormatString=|
      | %<ID>
      | %<Vbase>V
      | %<VLF>pu
      | %<angleLF>deg.
      | %<Name>
  bus40 : powerlib/Measurements/Load Flow Bus  LConnTagsString=a  ID=bus40  Vbase=110000  Vref=1  Vangle=0  VLF=1  angleLF=0
      settings: AttributesFormatString=|
      | %<ID>
      | %<Vbase>V
      | %<VLF>pu
      | %<angleLF>deg.
      | %<Name>
  bus41 : powerlib/Measurements/Load Flow Bus  LConnTagsString=a  ID=bus41  Vbase=110000  Vref=1  Vangle=0  VLF=1  angleLF=0
      settings: AttributesFormatString=|
      | %<ID>
      | %<Vbase>V
      | %<VLF>pu
      | %<angleLF>deg.
      | %<Name>
  bus42 : powerlib/Measurements/Load Flow Bus  LConnTagsString=a  ID=bus42  Vbase=110000  Vref=1  Vangle=0  VLF=1  angleLF=0
      settings: AttributesFormatString=|
      | %<ID>
      | %<Vbase>V
      | %<VLF>pu
      | %<angleLF>deg.
      | %<Name>
  bus43 : powerlib/Measurements/Load Flow Bus  LConnTagsString=a  ID=bus43  Vbase=110000  Vref=1  Vangle=0  VLF=1  angleLF=0
      settings: AttributesFormatString=|
      | %<ID>
      | %<Vbase>V
      | %<VLF>pu
      | %<angleLF>deg.
      | %<Name>
  bus44 : powerlib/Measurements/Load Flow Bus  LConnTagsString=a  ID=bus44  Vbase=110000  Vref=1  Vangle=0  VLF=1  angleLF=0
      settings: AttributesFormatString=|
      | %<ID>
      | %<Vbase>V
      | %<VLF>pu
      | %<angleLF>deg.
      | %<Name>
  bus45 : powerlib/Measurements/Load Flow Bus  LConnTagsString=a  ID=bus45  Vbase=110000  Vref=1  Vangle=0  VLF=1  angleLF=0
      settings: AttributesFormatString=|
      | %<ID>
      | %<Vbase>V
      | %<VLF>pu
      | %<angleLF>deg.
      | %<Name>
  bus46 : powerlib/Measurements/Load Flow Bus  LConnTagsString=a  ID=bus46  Vbase=110000  Vref=1  Vangle=0  VLF=1  angleLF=0
      settings: AttributesFormatString=|
      | %<ID>
      | %<Vbase>V
      | %<VLF>pu
      | %<angleLF>deg.
      | %<Name>
  bus47 : powerlib/Measurements/Load Flow Bus  LConnTagsString=a  ID=bus47  Vbase=110000  Vref=1  Vangle=0  VLF=1  angleLF=0
      settings: AttributesFormatString=|
      | %<ID>
      | %<Vbase>V
      | %<VLF>pu
      | %<angleLF>deg.
      | %<Name>
  bus48 : powerlib/Measurements/Load Flow Bus  LConnTagsString=a  ID=bus48  Vbase=110000  Vref=1  Vangle=0  VLF=1  angleLF=0
      settings: AttributesFormatString=|
      | %<ID>
      | %<Vbase>V
      | %<VLF>pu
      | %<angleLF>deg.
      | %<Name>
  bus49 : powerlib/Measurements/Load Flow Bus  LConnTagsString=a  ID=bus49  Vbase=110000  Vref=1  Vangle=0  VLF=1  angleLF=0
      settings: AttributesFormatString=|
      | %<ID>
      | %<Vbase>V
      | %<VLF>pu
      | %<angleLF>deg.
      | %<Name>
  bus5 : powerlib/Measurements/Load Flow Bus  LConnTagsString=a  ID=bus5  Vbase=110000  Vref=1  Vangle=0  VLF=1  angleLF=0
      settings: AttributesFormatString=|
      | %<ID>
      | %<Vbase>V
      | %<VLF>pu
      | %<angleLF>deg.
      | %<Name>
  bus50 : powerlib/Measurements/Load Flow Bus  LConnTagsString=a  ID=bus50  Vbase=110000  Vref=1  Vangle=0  VLF=1  angleLF=0
      settings: AttributesFormatString=|
      | %<ID>
      | %<Vbase>V
      | %<VLF>pu
      | %<angleLF>deg.
      | %<Name>
  bus51 : powerlib/Measurements/Load Flow Bus  LConnTagsString=a  ID=bus51  Vbase=110000  Vref=1  Vangle=0  VLF=1  angleLF=0
      settings: AttributesFormatString=|
      | %<ID>
      | %<Vbase>V
      | %<VLF>pu
      | %<angleLF>deg.
      | %<Name>
  bus52 : powerlib/Measurements/Load Flow Bus  LConnTagsString=a  ID=bus52  Vbase=110000  Vref=1  Vangle=0  VLF=1  angleLF=0
      settings: AttributesFormatString=|
      | %<ID>
      | %<Vbase>V
      | %<VLF>pu
      | %<angleLF>deg.
      | %<Name>
  bus53 : powerlib/Measurements/Load Flow Bus  LConnTagsString=a  ID=bus53  Vbase=110000  Vref=1  Vangle=0  VLF=1  angleLF=0
      settings: AttributesFormatString=|
      | %<ID>
      | %<Vbase>V
      | %<VLF>pu
      | %<angleLF>deg.
      | %<Name>
  bus54 : powerlib/Measurements/Load Flow Bus  LConnTagsString=a  ID=bus54  Vbase=110000  Vref=1  Vangle=0  VLF=1  angleLF=0
      settings: AttributesFormatString=|
      | %<ID>
      | %<Vbase>V
      | %<VLF>pu
      | %<angleLF>deg.
      | %<Name>
  bus55 : powerlib/Measurements/Load Flow Bus  LConnTagsString=a  ID=bus55  Vbase=110000  Vref=1  Vangle=0  VLF=1  angleLF=0
      settings: AttributesFormatString=|
      | %<ID>
      | %<Vbase>V
      | %<VLF>pu
      | %<angleLF>deg.
      | %<Name>
  bus56 : powerlib/Measurements/Load Flow Bus  LConnTagsString=a  ID=bus56  Vbase=110000  Vref=1  Vangle=0  VLF=1  angleLF=0
      settings: AttributesFormatString=|
      | %<ID>
      | %<Vbase>V
      | %<VLF>pu
      | %<angleLF>deg.
      | %<Name>
  bus57 : powerlib/Measurements/Load Flow Bus  LConnTagsString=a  ID=bus57  Vbase=110000  Vref=1  Vangle=0  VLF=1  angleLF=0
      settings: AttributesFormatString=|
      | %<ID>
      | %<Vbase>V
      | %<VLF>pu
      | %<angleLF>deg.
      | %<Name>
  bus58 : powerlib/Measurements/Load Flow Bus  LConnTagsString=a  ID=bus58  Vbase=110000  Vref=1  Vangle=0  VLF=1  angleLF=0
      settings: AttributesFormatString=|
      | %<ID>
      | %<Vbase>V
      | %<VLF>pu
      | %<angleLF>deg.
      | %<Name>
  bus59 : powerlib/Measurements/Load Flow Bus  LConnTagsString=a  ID=bus59  Vbase=110000  Vref=1  Vangle=0  VLF=1  angleLF=0
      settings: AttributesFormatString=|
      | %<ID>
      | %<Vbase>V
      | %<VLF>pu
      | %<angleLF>deg.
      | %<Name>
  bus6 : powerlib/Measurements/Load Flow Bus  LConnTagsString=a  ID=bus6  Vbase=110000  Vref=1  Vangle=0  VLF=1  angleLF=0
      settings: AttributesFormatString=|
      | %<ID>
      | %<Vbase>V
      | %<VLF>pu
      | %<angleLF>deg.
      | %<Name>
  bus60 : powerlib/Measurements/Load Flow Bus  LConnTagsString=a  ID=bus60  Vbase=110000  Vref=1  Vangle=0  VLF=1  angleLF=0
      settings: AttributesFormatString=|
      | %<ID>
      | %<Vbase>V
      | %<VLF>pu
      | %<angleLF>deg.
      | %<Name>
  bus61 : powerlib/Measurements/Load Flow Bus  LConnTagsString=a  ID=bus61  Vbase=110000  Vref=1  Vangle=0  VLF=1  angleLF=0
      settings: AttributesFormatString=|
      | %<ID>
      | %<Vbase>V
      | %<VLF>pu
      | %<angleLF>deg.
      | %<Name>
  bus62 : powerlib/Measurements/Load Flow Bus  LConnTagsString=a  ID=bus62  Vbase=110000  Vref=1  Vangle=0  VLF=1  angleLF=0
      settings: AttributesFormatString=|
      | %<ID>
      | %<Vbase>V
      | %<VLF>pu
      | %<angleLF>deg.
      | %<Name>
  bus63 : powerlib/Measurements/Load Flow Bus  LConnTagsString=a  ID=bus63  Vbase=110000  Vref=1  Vangle=0  VLF=1  angleLF=0
      settings: AttributesFormatString=|
      | %<ID>
      | %<Vbase>V
      | %<VLF>pu
      | %<angleLF>deg.
      | %<Name>
  bus64 : powerlib/Measurements/Load Flow Bus  LConnTagsString=a  ID=bus64  Vbase=110000  Vref=1  Vangle=0  VLF=1  angleLF=0
      settings: AttributesFormatString=|
      | %<ID>
      | %<Vbase>V
      | %<VLF>pu
      | %<angleLF>deg.
      | %<Name>
  bus65 : powerlib/Measurements/Load Flow Bus  LConnTagsString=a  ID=bus65  Vbase=110000  Vref=1  Vangle=0  VLF=1  angleLF=0
      settings: AttributesFormatString=|
      | %<ID>
      | %<Vbase>V
      | %<VLF>pu
      | %<angleLF>deg.
      | %<Name>
  bus66 : powerlib/Measurements/Load Flow Bus  LConnTagsString=a  ID=bus66  Vbase=110000  Vref=1  Vangle=0  VLF=1  angleLF=0
      settings: AttributesFormatString=|
      | %<ID>
      | %<Vbase>V
      | %<VLF>pu
      | %<angleLF>deg.
      | %<Name>
  bus67 : powerlib/Measurements/Load Flow Bus  LConnTagsString=a  ID=bus67  Vbase=110000  Vref=1  Vangle=0  VLF=1  angleLF=0
      settings: AttributesFormatString=|
      | %<ID>
      | %<Vbase>V
      | %<VLF>pu
      | %<angleLF>deg.
      | %<Name>
  bus68 : powerlib/Measurements/Load Flow Bus  LConnTagsString=a  ID=bus68  Vbase=110000  Vref=1  Vangle=0  VLF=1  angleLF=0
      settings: AttributesFormatString=|
      | %<ID>
      | %<Vbase>V
      | %<VLF>pu
      | %<angleLF>deg.
      | %<Name>
  bus69 : powerlib/Measurements/Load Flow Bus  LConnTagsString=a  ID=bus69  Vbase=110000  Vref=1  Vangle=0  VLF=1  angleLF=0
      settings: AttributesFormatString=|
      | %<ID>
      | %<Vbase>V
      | %<VLF>pu
      | %<angleLF>deg.
      | %<Name>
  bus7 : powerlib/Measurements/Load Flow Bus  LConnTagsString=a  ID=bus7  Vbase=110000  Vref=1  Vangle=0  VLF=1  angleLF=0
      settings: AttributesFormatString=|
      | %<ID>
      | %<Vbase>V
      | %<VLF>pu
      | %<angleLF>deg.
      | %<Name>
  bus70 : powerlib/Measurements/Load Flow Bus  LConnTagsString=a  ID=bus70  Vbase=110000  Vref=1  Vangle=0  VLF=1  angleLF=0
      settings: AttributesFormatString=|
      | %<ID>
      | %<Vbase>V
      | %<VLF>pu
      | %<angleLF>deg.
      | %<Name>
  bus71 : powerlib/Measurements/Load Flow Bus  LConnTagsString=a  ID=bus71  Vbase=110000  Vref=1  Vangle=0  VLF=1  angleLF=0
      settings: AttributesFormatString=|
      | %<ID>
      | %<Vbase>V
      | %<VLF>pu
      | %<angleLF>deg.
      | %<Name>
  bus72 : powerlib/Measurements/Load Flow Bus  LConnTagsString=a  ID=bus72  Vbase=110000  Vref=1  Vangle=0  VLF=1  angleLF=0
      settings: AttributesFormatString=|
      | %<ID>
      | %<Vbase>V
      | %<VLF>pu
      | %<angleLF>deg.
      | %<Name>
  bus73 : powerlib/Measurements/Load Flow Bus  LConnTagsString=a  ID=bus73  Vbase=110000  Vref=1  Vangle=0  VLF=1  angleLF=0
      settings: AttributesFormatString=|
      | %<ID>
      | %<Vbase>V
      | %<VLF>pu
      | %<angleLF>deg.
      | %<Name>
  bus74 : powerlib/Measurements/Load Flow Bus  LConnTagsString=a  ID=bus74  Vbase=110000  Vref=1  Vangle=0  VLF=1  angleLF=0
      settings: AttributesFormatString=|
      | %<ID>
      | %<Vbase>V
      | %<VLF>pu
      | %<angleLF>deg.
      | %<Name>
  bus75 : powerlib/Measurements/Load Flow Bus  LConnTagsString=a  ID=bus75  Vbase=110000  Vref=1  Vangle=0  VLF=1  angleLF=0
      settings: AttributesFormatString=|
      | %<ID>
      | %<Vbase>V
      | %<VLF>pu
      | %<angleLF>deg.
      | %<Name>
  bus76 : powerlib/Measurements/Load Flow Bus  LConnTagsString=a  ID=bus76  Vbase=110000  Vref=1  Vangle=0  VLF=1  angleLF=0
      settings: AttributesFormatString=|
      | %<ID>
      | %<Vbase>V
      | %<VLF>pu
      | %<angleLF>deg.
      | %<Name>
  bus77 : powerlib/Measurements/Load Flow Bus  LConnTagsString=a  ID=bus77  Vbase=110000  Vref=1  Vangle=0  VLF=1  angleLF=0
      settings: AttributesFormatString=|
      | %<ID>
      | %<Vbase>V
      | %<VLF>pu
      | %<angleLF>deg.
      | %<Name>
  bus78 : powerlib/Measurements/Load Flow Bus  LConnTagsString=a  ID=bus78  Vbase=110000  Vref=1  Vangle=0  VLF=1  angleLF=0
      settings: AttributesFormatString=|
      | %<ID>
      | %<Vbase>V
      | %<VLF>pu
      | %<angleLF>deg.
      | %<Name>
  bus79 : powerlib/Measurements/Load Flow Bus  LConnTagsString=a  ID=bus79  Vbase=110000  Vref=1  Vangle=0  VLF=1  angleLF=0
      settings: AttributesFormatString=|
      | %<ID>
      | %<Vbase>V
      | %<VLF>pu
      | %<angleLF>deg.
      | %<Name>
  bus8 : powerlib/Measurements/Load Flow Bus  LConnTagsString=a  ID=bus8  Vbase=110000  Vref=1  Vangle=0  VLF=1  angleLF=0
      settings: AttributesFormatString=|
      | %<ID>
      | %<Vbase>V
      | %<VLF>pu
      | %<angleLF>deg.
      | %<Name>
  bus80 : powerlib/Measurements/Load Flow Bus  LConnTagsString=a  ID=bus80  Vbase=110000  Vref=1  Vangle=0  VLF=1  angleLF=0
      settings: AttributesFormatString=|
      | %<ID>
      | %<Vbase>V
      | %<VLF>pu
      | %<angleLF>deg.
      | %<Name>
  bus81 : powerlib/Measurements/Load Flow Bus  LConnTagsString=a  ID=bus81  Vbase=110000  Vref=1  Vangle=0  VLF=1  angleLF=0
      settings: AttributesFormatString=|
      | %<ID>
      | %<Vbase>V
      | %<VLF>pu
      | %<angleLF>deg.
      | %<Name>
  bus82 : powerlib/Measurements/Load Flow Bus  LConnTagsString=a  ID=bus82  Vbase=110000  Vref=1  Vangle=0  VLF=1  angleLF=0
      settings: AttributesFormatString=|
      | %<ID>
      | %<Vbase>V
      | %<VLF>pu
      | %<angleLF>deg.
      | %<Name>
  bus83 : powerlib/Measurements/Load Flow Bus  LConnTagsString=a  ID=bus83  Vbase=110000  Vref=1  Vangle=0  VLF=1  angleLF=0
      settings: AttributesFormatString=|
      | %<ID>
      | %<Vbase>V
      | %<VLF>pu
      | %<angleLF>deg.
      | %<Name>
  bus84 : powerlib/Measurements/Load Flow Bus  LConnTagsString=a  ID=bus84  Vbase=110000  Vref=1  Vangle=0  VLF=1  angleLF=0
      settings: AttributesFormatString=|
      | %<ID>
      | %<Vbase>V
      | %<VLF>pu
      | %<angleLF>deg.
      | %<Name>
  bus85 : powerlib/Measurements/Load Flow Bus  LConnTagsString=a  ID=bus85  Vbase=110000  Vref=1  Vangle=0  VLF=1  angleLF=0
      settings: AttributesFormatString=|
      | %<ID>
      | %<Vbase>V
      | %<VLF>pu
      | %<angleLF>deg.
      | %<Name>
  bus86 : powerlib/Measurements/Load Flow Bus  LConnTagsString=a  ID=bus86  Vbase=110000  Vref=1  Vangle=0  VLF=1  angleLF=0
      settings: AttributesFormatString=|
      | %<ID>
      | %<Vbase>V
      | %<VLF>pu
      | %<angleLF>deg.
      | %<Name>
  bus87 : powerlib/Measurements/Load Flow Bus  LConnTagsString=a  ID=bus87  Vbase=110000  Vref=1  Vangle=0  VLF=1  angleLF=0
      settings: AttributesFormatString=|
      | %<ID>
      | %<Vbase>V
      | %<VLF>pu
      | %<angleLF>deg.
      | %<Name>
  bus88 : powerlib/Measurements/Load Flow Bus  LConnTagsString=a  ID=bus88  Vbase=110000  Vref=1  Vangle=0  VLF=1  angleLF=0
      settings: AttributesFormatString=|
      | %<ID>
      | %<Vbase>V
      | %<VLF>pu
      | %<angleLF>deg.
      | %<Name>
  bus89 : powerlib/Measurements/Load Flow Bus  LConnTagsString=a  ID=bus89  Vbase=110000  Vref=1  Vangle=0  VLF=1  angleLF=0
      settings: AttributesFormatString=|
      | %<ID>
      | %<Vbase>V
      | %<VLF>pu
      | %<angleLF>deg.
      | %<Name>
  bus9 : powerlib/Measurements/Load Flow Bus  LConnTagsString=a  ID=bus9  Vbase=110000  Vref=1  Vangle=0  VLF=1  angleLF=0
      settings: AttributesFormatString=|
      | %<ID>
      | %<Vbase>V
      | %<VLF>pu
      | %<angleLF>deg.
      | %<Name>
  bus90 : powerlib/Measurements/Load Flow Bus  LConnTagsString=a  ID=bus90  Vbase=110000  Vref=1  Vangle=0  VLF=1  angleLF=0
      settings: AttributesFormatString=|
      | %<ID>
      | %<Vbase>V
      | %<VLF>pu
      | %<angleLF>deg.
      | %<Name>
  bus91 : powerlib/Measurements/Load Flow Bus  LConnTagsString=a  ID=bus91  Vbase=110000  Vref=1  Vangle=0  VLF=1  angleLF=0
      settings: AttributesFormatString=|
      | %<ID>
      | %<Vbase>V
      | %<VLF>pu
      | %<angleLF>deg.
      | %<Name>
  bus92 : powerlib/Measurements/Load Flow Bus  LConnTagsString=a  ID=bus92  Vbase=110000  Vref=1  Vangle=0  VLF=1  angleLF=0
      settings: AttributesFormatString=|
      | %<ID>
      | %<Vbase>V
      | %<VLF>pu
      | %<angleLF>deg.
      | %<Name>
  bus93 : powerlib/Measurements/Load Flow Bus  LConnTagsString=a  ID=bus93  Vbase=110000  Vref=1  Vangle=0  VLF=1  angleLF=0
      settings: AttributesFormatString=|
      | %<ID>
      | %<Vbase>V
      | %<VLF>pu
      | %<angleLF>deg.
      | %<Name>
  bus94 : powerlib/Measurements/Load Flow Bus  LConnTagsString=a  ID=bus94  Vbase=110000  Vref=1  Vangle=0  VLF=1  angleLF=0
      settings: AttributesFormatString=|
      | %<ID>
      | %<Vbase>V
      | %<VLF>pu
      | %<angleLF>deg.
      | %<Name>
  bus95 : powerlib/Measurements/Load Flow Bus  LConnTagsString=a  ID=bus95  Vbase=110000  Vref=1  Vangle=0  VLF=1  angleLF=0
      settings: AttributesFormatString=|
      | %<ID>
      | %<Vbase>V
      | %<VLF>pu
      | %<angleLF>deg.
      | %<Name>
  bus96 : powerlib/Measurements/Load Flow Bus  LConnTagsString=a  ID=bus96  Vbase=110000  Vref=1  Vangle=0  VLF=1  angleLF=0
      settings: AttributesFormatString=|
      | %<ID>
      | %<Vbase>V
      | %<VLF>pu
      | %<angleLF>deg.
      | %<Name>
  bus97 : powerlib/Measurements/Load Flow Bus  LConnTagsString=a  ID=bus97  Vbase=110000  Vref=1  Vangle=0  VLF=1  angleLF=0
      settings: AttributesFormatString=|
      | %<ID>
      | %<Vbase>V
      | %<VLF>pu
      | %<angleLF>deg.
      | %<Name>
  bus98 : powerlib/Measurements/Load Flow Bus  LConnTagsString=a  ID=bus98  Vbase=110000  Vref=1  Vangle=0  VLF=1  angleLF=0
      settings: AttributesFormatString=|
      | %<ID>
      | %<Vbase>V
      | %<VLF>pu
      | %<angleLF>deg.
      | %<Name>
  bus99 : powerlib/Measurements/Load Flow Bus  LConnTagsString=a  ID=bus99  Vbase=110000  Vref=1  Vangle=0  VLF=1  angleLF=0
      settings: AttributesFormatString=|
      | %<ID>
      | %<Vbase>V
      | %<VLF>pu
      | %<angleLF>deg.
      | %<Name>
